simulink model "w3_warplab_buffers"  (Simulink 7.7)
settings: Solver=VariableStepDiscrete  SolverMode=SingleTasking  StartTime=0.0  StopTime=100  RelTol=1e-3
InitFcn:
  | w3_warplab_buffers_init
StartFcn:
  | w3_warplab_buffers_init
values from neighbouring files (symbols this model uses):
  NumSamps_Rx_IQ = 2^15    (= 32768)    [w3_warplab_buffers_init.m]
  NumSamps_Rx_RSSI = 2^13    (= 8192)    [w3_warplab_buffers_init.m]
  NumSamps_Tx_IQ = 2^15    (= 32768)    [w3_warplab_buffers_init.m]
undefined symbols (not defined in the file or in its folder): gcbh, xlBlockLoadCallback, xlGetNormalizedPeriod
libraries: xbsIndex_r4 x453, xbsEDKLib_r4 x1
(part 2 of 5)

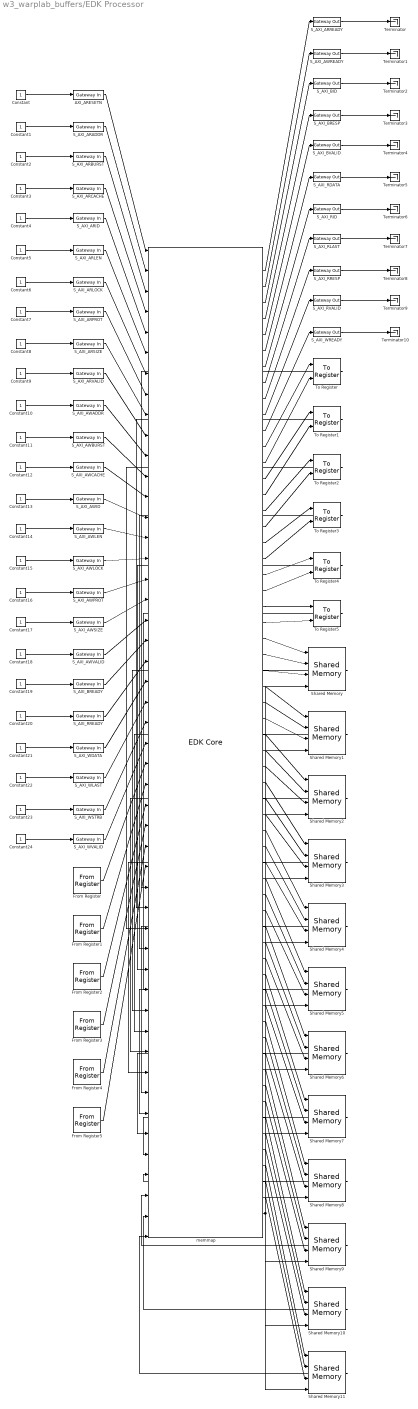
== system w3_warplab_buffers/EDK Processor ==
  AXI_ARESETN : xbsIndex_r4/Gateway In  gui_display_data_type=Fixed-point  arith_type=Boolean  n_bits=16  bin_pt=14  preci_type=Single  exp_width=8  frac_width=24  quantization="Round  (unbiased: +/- Inf)"  overflow=Saturate  period=xlGetNormalizedPeriod()  dbl_ovrd=off  timing_constraint=None  locs_specified=off  LOCs={}  UseAsADC=off  ADCChannel='1'  inherit_from_input=off  hdl_port=on  block_type=gatewayin
  Constant{,1..24} (25 alike) : Constant
  From Register : xbsIndex_r4/From Register  shared_memory_name='BUFF_SIZES'  init=0  period=xlGetNormalizedPeriod()  ownership=Owned and initialized elsewhere  gui_display_data_type=Fixed-point  arith_type=Unsigned  n_bits=32  bin_pt=0  preci_type=Single  dbl_ovrd=off  block_type=fromreg
      settings: AttributesFormatString=<< %<shared_memory_name> >>  infoedit="Register block that reads data to a shared memory register.  Delay of one sample period."
  From Register1 : xbsIndex_r4/From Register  shared_memory_name='DESIGN_VER'  init=0  period=xlGetNormalizedPeriod()  ownership=Owned and initialized elsewhere  gui_display_data_type=Fixed-point  arith_type=Unsigned  n_bits=32  bin_pt=0  preci_type=Single  dbl_ovrd=off  block_type=fromreg
      settings: AttributesFormatString=<< %<shared_memory_name> >>  infoedit="Register block that reads data to a shared memory register.  Delay of one sample period."
  From Register2 : xbsIndex_r4/From Register  shared_memory_name='STATUS'  init=0  period=xlGetNormalizedPeriod()  ownership=Owned and initialized elsewhere  gui_display_data_type=Fixed-point  arith_type=Unsigned  n_bits=2  bin_pt=0  preci_type=Single  dbl_ovrd=off  block_type=fromreg
      settings: AttributesFormatString=<< %<shared_memory_name> >>  infoedit="Register block that reads data to a shared memory register.  Delay of one sample period."
  From Register3 : xbsIndex_r4/From Register  shared_memory_name='RFCD_AGCDoneRSSI'  init=0  period=xlGetNormalizedPeriod()  ownership=Owned and initialized elsewhere  gui_display_data_type=Fixed-point  arith_type=Unsigned  n_bits=32  bin_pt=0  preci_type=Single  dbl_ovrd=off  block_type=fromreg
      settings: AttributesFormatString=<< %<shared_memory_name> >>  infoedit="Register block that reads data to a shared memory register.  Delay of one sample period."
  From Register4 : xbsIndex_r4/From Register  shared_memory_name='RFAB_AGCDoneRSSI'  init=0  period=xlGetNormalizedPeriod()  ownership=Owned and initialized elsewhere  gui_display_data_type=Fixed-point  arith_type=Unsigned  n_bits=32  bin_pt=0  preci_type=Single  dbl_ovrd=off  block_type=fromreg
      settings: AttributesFormatString=<< %<shared_memory_name> >>  infoedit="Register block that reads data to a shared memory register.  Delay of one sample period."
  From Register5 : xbsIndex_r4/From Register  shared_memory_name='AGCDoneAddr'  init=0  period=xlGetNormalizedPeriod()  ownership=Owned and initialized elsewhere  gui_display_data_type=Fixed-point  arith_type=Unsigned  n_bits=32  bin_pt=0  preci_type=Single  dbl_ovrd=off  block_type=fromreg
      settings: AttributesFormatString=<< %<shared_memory_name> >>  infoedit="Register block that reads data to a shared memory register.  Delay of one sample period."
  S_AXI_ARADDR : xbsIndex_r4/Gateway In  gui_display_data_type=Fixed-point  arith_type=Unsigned  n_bits=32  bin_pt=0  preci_type=Single  exp_width=8  frac_width=24  quantization="Round  (unbiased: +/- Inf)"  overflow=Saturate  period=xlGetNormalizedPeriod()  dbl_ovrd=off  timing_constraint=None  locs_specified=off  LOCs={}  UseAsADC=off  ADCChannel='1'  inherit_from_input=off  hdl_port=on  block_type=gatewayin
  S_AXI_ARBURST : xbsIndex_r4/Gateway In  gui_display_data_type=Fixed-point  arith_type=Unsigned  n_bits=2  bin_pt=0  preci_type=Single  exp_width=8  frac_width=24  quantization="Round  (unbiased: +/- Inf)"  overflow=Saturate  period=xlGetNormalizedPeriod()  dbl_ovrd=off  timing_constraint=None  locs_specified=off  LOCs={}  UseAsADC=off  ADCChannel='1'  inherit_from_input=off  hdl_port=on  block_type=gatewayin
  S_AXI_ARCACHE : xbsIndex_r4/Gateway In  gui_display_data_type=Fixed-point  arith_type=Unsigned  n_bits=4  bin_pt=0  preci_type=Single  exp_width=8  frac_width=24  quantization="Round  (unbiased: +/- Inf)"  overflow=Saturate  period=xlGetNormalizedPeriod()  dbl_ovrd=off  timing_constraint=None  locs_specified=off  LOCs={}  UseAsADC=off  ADCChannel='1'  inherit_from_input=off  hdl_port=on  block_type=gatewayin
  S_AXI_ARID : xbsIndex_r4/Gateway In  gui_display_data_type=Fixed-point  arith_type=Unsigned  n_bits=8  bin_pt=0  preci_type=Single  exp_width=8  frac_width=24  quantization="Round  (unbiased: +/- Inf)"  overflow=Saturate  period=xlGetNormalizedPeriod()  dbl_ovrd=off  timing_constraint=None  locs_specified=off  LOCs={}  UseAsADC=off  ADCChannel='1'  inherit_from_input=off  hdl_port=on  block_type=gatewayin
  S_AXI_ARLEN : xbsIndex_r4/Gateway In  gui_display_data_type=Fixed-point  arith_type=Unsigned  n_bits=8  bin_pt=0  preci_type=Single  exp_width=8  frac_width=24  quantization="Round  (unbiased: +/- Inf)"  overflow=Saturate  period=xlGetNormalizedPeriod()  dbl_ovrd=off  timing_constraint=None  locs_specified=off  LOCs={}  UseAsADC=off  ADCChannel='1'  inherit_from_input=off  hdl_port=on  block_type=gatewayin
  S_AXI_ARLOCK : xbsIndex_r4/Gateway In  gui_display_data_type=Fixed-point  arith_type=Unsigned  n_bits=2  bin_pt=0  preci_type=Single  exp_width=8  frac_width=24  quantization="Round  (unbiased: +/- Inf)"  overflow=Saturate  period=xlGetNormalizedPeriod()  dbl_ovrd=off  timing_constraint=None  locs_specified=off  LOCs={}  UseAsADC=off  ADCChannel='1'  inherit_from_input=off  hdl_port=on  block_type=gatewayin
  S_AXI_ARPROT : xbsIndex_r4/Gateway In  gui_display_data_type=Fixed-point  arith_type=Unsigned  n_bits=3  bin_pt=0  preci_type=Single  exp_width=8  frac_width=24  quantization="Round  (unbiased: +/- Inf)"  overflow=Saturate  period=xlGetNormalizedPeriod()  dbl_ovrd=off  timing_constraint=None  locs_specified=off  LOCs={}  UseAsADC=off  ADCChannel='1'  inherit_from_input=off  hdl_port=on  block_type=gatewayin
  S_AXI_ARREADY : xbsIndex_r4/Gateway Out  inherit_from_input=off  hdl_port=on  timing_constraint=None  locs_specified=off  LOCs={}  UseAsDAC=off  DACChannel='1'  block_type=gatewayout
  S_AXI_ARSIZE : xbsIndex_r4/Gateway In  gui_display_data_type=Fixed-point  arith_type=Unsigned  n_bits=3  bin_pt=0  preci_type=Single  exp_width=8  frac_width=24  quantization="Round  (unbiased: +/- Inf)"  overflow=Saturate  period=xlGetNormalizedPeriod()  dbl_ovrd=off  timing_constraint=None  locs_specified=off  LOCs={}  UseAsADC=off  ADCChannel='1'  inherit_from_input=off  hdl_port=on  block_type=gatewayin
  S_AXI_ARVALID : xbsIndex_r4/Gateway In  gui_display_data_type=Fixed-point  arith_type=Boolean  n_bits=16  bin_pt=14  preci_type=Single  exp_width=8  frac_width=24  quantization="Round  (unbiased: +/- Inf)"  overflow=Saturate  period=xlGetNormalizedPeriod()  dbl_ovrd=off  timing_constraint=None  locs_specified=off  LOCs={}  UseAsADC=off  ADCChannel='1'  inherit_from_input=off  hdl_port=on  block_type=gatewayin
  S_AXI_AWADDR : xbsIndex_r4/Gateway In  gui_display_data_type=Fixed-point  arith_type=Unsigned  n_bits=32  bin_pt=0  preci_type=Single  exp_width=8  frac_width=24  quantization="Round  (unbiased: +/- Inf)"  overflow=Saturate  period=xlGetNormalizedPeriod()  dbl_ovrd=off  timing_constraint=None  locs_specified=off  LOCs={}  UseAsADC=off  ADCChannel='1'  inherit_from_input=off  hdl_port=on  block_type=gatewayin
  S_AXI_AWBURST : xbsIndex_r4/Gateway In  gui_display_data_type=Fixed-point  arith_type=Unsigned  n_bits=2  bin_pt=0  preci_type=Single  exp_width=8  frac_width=24  quantization="Round  (unbiased: +/- Inf)"  overflow=Saturate  period=xlGetNormalizedPeriod()  dbl_ovrd=off  timing_constraint=None  locs_specified=off  LOCs={}  UseAsADC=off  ADCChannel='1'  inherit_from_input=off  hdl_port=on  block_type=gatewayin
  S_AXI_AWCACHE : xbsIndex_r4/Gateway In  gui_display_data_type=Fixed-point  arith_type=Unsigned  n_bits=4  bin_pt=0  preci_type=Single  exp_width=8  frac_width=24  quantization="Round  (unbiased: +/- Inf)"  overflow=Saturate  period=xlGetNormalizedPeriod()  dbl_ovrd=off  timing_constraint=None  locs_specified=off  LOCs={}  UseAsADC=off  ADCChannel='1'  inherit_from_input=off  hdl_port=on  block_type=gatewayin
  S_AXI_AWID : xbsIndex_r4/Gateway In  gui_display_data_type=Fixed-point  arith_type=Unsigned  n_bits=8  bin_pt=0  preci_type=Single  exp_width=8  frac_width=24  quantization="Round  (unbiased: +/- Inf)"  overflow=Saturate  period=xlGetNormalizedPeriod()  dbl_ovrd=off  timing_constraint=None  locs_specified=off  LOCs={}  UseAsADC=off  ADCChannel='1'  inherit_from_input=off  hdl_port=on  block_type=gatewayin
  S_AXI_AWLEN : xbsIndex_r4/Gateway In  gui_display_data_type=Fixed-point  arith_type=Unsigned  n_bits=8  bin_pt=0  preci_type=Single  exp_width=8  frac_width=24  quantization="Round  (unbiased: +/- Inf)"  overflow=Saturate  period=xlGetNormalizedPeriod()  dbl_ovrd=off  timing_constraint=None  locs_specified=off  LOCs={}  UseAsADC=off  ADCChannel='1'  inherit_from_input=off  hdl_port=on  block_type=gatewayin
  S_AXI_AWLOCK : xbsIndex_r4/Gateway In  gui_display_data_type=Fixed-point  arith_type=Unsigned  n_bits=2  bin_pt=0  preci_type=Single  exp_width=8  frac_width=24  quantization="Round  (unbiased: +/- Inf)"  overflow=Saturate  period=xlGetNormalizedPeriod()  dbl_ovrd=off  timing_constraint=None  locs_specified=off  LOCs={}  UseAsADC=off  ADCChannel='1'  inherit_from_input=off  hdl_port=on  block_type=gatewayin
  S_AXI_AWPROT : xbsIndex_r4/Gateway In  gui_display_data_type=Fixed-point  arith_type=Unsigned  n_bits=3  bin_pt=0  preci_type=Single  exp_width=8  frac_width=24  quantization="Round  (unbiased: +/- Inf)"  overflow=Saturate  period=xlGetNormalizedPeriod()  dbl_ovrd=off  timing_constraint=None  locs_specified=off  LOCs={}  UseAsADC=off  ADCChannel='1'  inherit_from_input=off  hdl_port=on  block_type=gatewayin
  S_AXI_AWREADY : xbsIndex_r4/Gateway Out  inherit_from_input=off  hdl_port=on  timing_constraint=None  locs_specified=off  LOCs={}  UseAsDAC=off  DACChannel='1'  block_type=gatewayout
  S_AXI_AWSIZE : xbsIndex_r4/Gateway In  gui_display_data_type=Fixed-point  arith_type=Unsigned  n_bits=3  bin_pt=0  preci_type=Single  exp_width=8  frac_width=24  quantization="Round  (unbiased: +/- Inf)"  overflow=Saturate  period=xlGetNormalizedPeriod()  dbl_ovrd=off  timing_constraint=None  locs_specified=off  LOCs={}  UseAsADC=off  ADCChannel='1'  inherit_from_input=off  hdl_port=on  block_type=gatewayin
  S_AXI_AWVALID : xbsIndex_r4/Gateway In  gui_display_data_type=Fixed-point  arith_type=Boolean  n_bits=16  bin_pt=14  preci_type=Single  exp_width=8  frac_width=24  quantization="Round  (unbiased: +/- Inf)"  overflow=Saturate  period=xlGetNormalizedPeriod()  dbl_ovrd=off  timing_constraint=None  locs_specified=off  LOCs={}  UseAsADC=off  ADCChannel='1'  inherit_from_input=off  hdl_port=on  block_type=gatewayin
  S_AXI_BID : xbsIndex_r4/Gateway Out  inherit_from_input=off  hdl_port=on  timing_constraint=None  locs_specified=off  LOCs={}  UseAsDAC=off  DACChannel='1'  block_type=gatewayout
  S_AXI_BREADY : xbsIndex_r4/Gateway In  gui_display_data_type=Fixed-point  arith_type=Boolean  n_bits=16  bin_pt=14  preci_type=Single  exp_width=8  frac_width=24  quantization="Round  (unbiased: +/- Inf)"  overflow=Saturate  period=xlGetNormalizedPeriod()  dbl_ovrd=off  timing_constraint=None  locs_specified=off  LOCs={}  UseAsADC=off  ADCChannel='1'  inherit_from_input=off  hdl_port=on  block_type=gatewayin
  S_AXI_BRESP : xbsIndex_r4/Gateway Out  inherit_from_input=off  hdl_port=on  timing_constraint=None  locs_specified=off  LOCs={}  UseAsDAC=off  DACChannel='1'  block_type=gatewayout
  S_AXI_BVALID : xbsIndex_r4/Gateway Out  inherit_from_input=off  hdl_port=on  timing_constraint=None  locs_specified=off  LOCs={}  UseAsDAC=off  DACChannel='1'  block_type=gatewayout
  S_AXI_RDATA : xbsIndex_r4/Gateway Out  inherit_from_input=off  hdl_port=on  timing_constraint=None  locs_specified=off  LOCs={}  UseAsDAC=off  DACChannel='1'  block_type=gatewayout
  S_AXI_RID : xbsIndex_r4/Gateway Out  inherit_from_input=off  hdl_port=on  timing_constraint=None  locs_specified=off  LOCs={}  UseAsDAC=off  DACChannel='1'  block_type=gatewayout
  S_AXI_RLAST : xbsIndex_r4/Gateway Out  inherit_from_input=off  hdl_port=on  timing_constraint=None  locs_specified=off  LOCs={}  UseAsDAC=off  DACChannel='1'  block_type=gatewayout
  S_AXI_RREADY : xbsIndex_r4/Gateway In  gui_display_data_type=Fixed-point  arith_type=Boolean  n_bits=16  bin_pt=14  preci_type=Single  exp_width=8  frac_width=24  quantization="Round  (unbiased: +/- Inf)"  overflow=Saturate  period=xlGetNormalizedPeriod()  dbl_ovrd=off  timing_constraint=None  locs_specified=off  LOCs={}  UseAsADC=off  ADCChannel='1'  inherit_from_input=off  hdl_port=on  block_type=gatewayin
  S_AXI_RRESP : xbsIndex_r4/Gateway Out  inherit_from_input=off  hdl_port=on  timing_constraint=None  locs_specified=off  LOCs={}  UseAsDAC=off  DACChannel='1'  block_type=gatewayout
  S_AXI_RVALID : xbsIndex_r4/Gateway Out  inherit_from_input=off  hdl_port=on  timing_constraint=None  locs_specified=off  LOCs={}  UseAsDAC=off  DACChannel='1'  block_type=gatewayout
  S_AXI_WDATA : xbsIndex_r4/Gateway In  gui_display_data_type=Fixed-point  arith_type=Unsigned  n_bits=32  bin_pt=0  preci_type=Single  exp_width=8  frac_width=24  quantization="Round  (unbiased: +/- Inf)"  overflow=Saturate  period=xlGetNormalizedPeriod()  dbl_ovrd=off  timing_constraint=None  locs_specified=off  LOCs={}  UseAsADC=off  ADCChannel='1'  inherit_from_input=off  hdl_port=on  block_type=gatewayin
  S_AXI_WLAST : xbsIndex_r4/Gateway In  gui_display_data_type=Fixed-point  arith_type=Boolean  n_bits=16  bin_pt=14  preci_type=Single  exp_width=8  frac_width=24  quantization="Round  (unbiased: +/- Inf)"  overflow=Saturate  period=xlGetNormalizedPeriod()  dbl_ovrd=off  timing_constraint=None  locs_specified=off  LOCs={}  UseAsADC=off  ADCChannel='1'  inherit_from_input=off  hdl_port=on  block_type=gatewayin
  S_AXI_WREADY : xbsIndex_r4/Gateway Out  inherit_from_input=off  hdl_port=on  timing_constraint=None  locs_specified=off  LOCs={}  UseAsDAC=off  DACChannel='1'  block_type=gatewayout
  S_AXI_WSTRB : xbsIndex_r4/Gateway In  gui_display_data_type=Fixed-point  arith_type=Unsigned  n_bits=4  bin_pt=0  preci_type=Single  exp_width=8  frac_width=24  quantization="Round  (unbiased: +/- Inf)"  overflow=Saturate  period=xlGetNormalizedPeriod()  dbl_ovrd=off  timing_constraint=None  locs_specified=off  LOCs={}  UseAsADC=off  ADCChannel='1'  inherit_from_input=off  hdl_port=on  block_type=gatewayin
  S_AXI_WVALID : xbsIndex_r4/Gateway In  gui_display_data_type=Fixed-point  arith_type=Boolean  n_bits=16  bin_pt=14  preci_type=Single  exp_width=8  frac_width=24  quantization="Round  (unbiased: +/- Inf)"  overflow=Saturate  period=xlGetNormalizedPeriod()  dbl_ovrd=off  timing_constraint=None  locs_specified=off  LOCs={}  UseAsADC=off  ADCChannel='1'  inherit_from_input=off  hdl_port=on  block_type=gatewayin
  Shared Memory : xbsIndex_r4/Shared Memory  shared_memory_name='RFD_IQ_Tx_Buffer'  depth=32768  ownership=Owned and Initialized Elsewhere  initVector=sin(pi*(0:15)/16)  en=on  mutex=Unprotected  mode=Read and Write  write_mode=Read Before Write  time_out=0  latency=1  explicit_data_type=off  gui_display_data_type=Fixed-point  arith_type=Unsigned  n_bits=32  bin_pt=0  preci_type=Single  implementation=Block RAM  use_rpm=off  block_type=shmem
      settings: AttributesFormatString=<< %<shared_memory_name> >>
  Shared Memory1 : xbsIndex_r4/Shared Memory  shared_memory_name='RFD_RSSI_Buffer'  depth=4096  ownership=Owned and Initialized Elsewhere  initVector=sin(pi*(0:15)/16)  en=on  mutex=Unprotected  mode=Read and Write  write_mode=Read Before Write  time_out=0  latency=1  explicit_data_type=off  gui_display_data_type=Fixed-point  arith_type=Unsigned  n_bits=32  bin_pt=0  preci_type=Single  implementation=Block RAM  use_rpm=off  block_type=shmem
      settings: AttributesFormatString=<< %<shared_memory_name> >>
  Shared Memory10 : xbsIndex_r4/Shared Memory  shared_memory_name='RFA_RSSI_Buffer'  depth=4096  ownership=Owned and Initialized Elsewhere  initVector=sin(pi*(0:15)/16)  en=on  mutex=Unprotected  mode=Read and Write  write_mode=Read Before Write  time_out=0  latency=1  explicit_data_type=off  gui_display_data_type=Fixed-point  arith_type=Unsigned  n_bits=32  bin_pt=0  preci_type=Single  implementation=Block RAM  use_rpm=off  block_type=shmem
      settings: AttributesFormatString=<< %<shared_memory_name> >>
  Shared Memory11 : xbsIndex_r4/Shared Memory  shared_memory_name='RFA_IQ_Rx_Buffer'  depth=32768  ownership=Owned and Initialized Elsewhere  initVector=sin(pi*(0:15)/16)  en=on  mutex=Unprotected  mode=Read and Write  write_mode=Read Before Write  time_out=0  latency=1  explicit_data_type=off  gui_display_data_type=Fixed-point  arith_type=Unsigned  n_bits=32  bin_pt=0  preci_type=Single  implementation=Block RAM  use_rpm=off  block_type=shmem
      settings: AttributesFormatString=<< %<shared_memory_name> >>
  Shared Memory2 : xbsIndex_r4/Shared Memory  shared_memory_name='RFD_IQ_Rx_Buffer'  depth=32768  ownership=Owned and Initialized Elsewhere  initVector=sin(pi*(0:15)/16)  en=on  mutex=Unprotected  mode=Read and Write  write_mode=Read Before Write  time_out=0  latency=1  explicit_data_type=off  gui_display_data_type=Fixed-point  arith_type=Unsigned  n_bits=32  bin_pt=0  preci_type=Single  implementation=Block RAM  use_rpm=off  block_type=shmem
      settings: AttributesFormatString=<< %<shared_memory_name> >>
  Shared Memory3 : xbsIndex_r4/Shared Memory  shared_memory_name='RFC_IQ_Tx_Buffer'  depth=32768  ownership=Owned and Initialized Elsewhere  initVector=sin(pi*(0:15)/16)  en=on  mutex=Unprotected  mode=Read and Write  write_mode=Read Before Write  time_out=0  latency=1  explicit_data_type=off  gui_display_data_type=Fixed-point  arith_type=Unsigned  n_bits=32  bin_pt=0  preci_type=Single  implementation=Block RAM  use_rpm=off  block_type=shmem
      settings: AttributesFormatString=<< %<shared_memory_name> >>
  Shared Memory4 : xbsIndex_r4/Shared Memory  shared_memory_name='RFC_RSSI_Buffer'  depth=4096  ownership=Owned and Initialized Elsewhere  initVector=sin(pi*(0:15)/16)  en=on  mutex=Unprotected  mode=Read and Write  write_mode=Read Before Write  time_out=0  latency=1  explicit_data_type=off  gui_display_data_type=Fixed-point  arith_type=Unsigned  n_bits=32  bin_pt=0  preci_type=Single  implementation=Block RAM  use_rpm=off  block_type=shmem
      settings: AttributesFormatString=<< %<shared_memory_name> >>
  Shared Memory5 : xbsIndex_r4/Shared Memory  shared_memory_name='RFC_IQ_Rx_Buffer'  depth=32768  ownership=Owned and Initialized Elsewhere  initVector=sin(pi*(0:15)/16)  en=on  mutex=Unprotected  mode=Read and Write  write_mode=Read Before Write  time_out=0  latency=1  explicit_data_type=off  gui_display_data_type=Fixed-point  arith_type=Unsigned  n_bits=32  bin_pt=0  preci_type=Single  implementation=Block RAM  use_rpm=off  block_type=shmem
      settings: AttributesFormatString=<< %<shared_memory_name> >>
  Shared Memory6 : xbsIndex_r4/Shared Memory  shared_memory_name='RFB_IQ_Tx_Buffer'  depth=32768  ownership=Owned and Initialized Elsewhere  initVector=sin(pi*(0:15)/16)  en=on  mutex=Unprotected  mode=Read and Write  write_mode=Read Before Write  time_out=0  latency=1  explicit_data_type=off  gui_display_data_type=Fixed-point  arith_type=Unsigned  n_bits=32  bin_pt=0  preci_type=Single  implementation=Block RAM  use_rpm=off  block_type=shmem
      settings: AttributesFormatString=<< %<shared_memory_name> >>
  Shared Memory7 : xbsIndex_r4/Shared Memory  shared_memory_name='RFB_RSSI_Buffer'  depth=4096  ownership=Owned and Initialized Elsewhere  initVector=sin(pi*(0:15)/16)  en=on  mutex=Unprotected  mode=Read and Write  write_mode=Read Before Write  time_out=0  latency=1  explicit_data_type=off  gui_display_data_type=Fixed-point  arith_type=Unsigned  n_bits=32  bin_pt=0  preci_type=Single  implementation=Block RAM  use_rpm=off  block_type=shmem
      settings: AttributesFormatString=<< %<shared_memory_name> >>
  Shared Memory8 : xbsIndex_r4/Shared Memory  shared_memory_name='RFB_IQ_Rx_Buffer'  depth=32768  ownership=Owned and Initialized Elsewhere  initVector=sin(pi*(0:15)/16)  en=on  mutex=Unprotected  mode=Read and Write  write_mode=Read Before Write  time_out=0  latency=1  explicit_data_type=off  gui_display_data_type=Fixed-point  arith_type=Unsigned  n_bits=32  bin_pt=0  preci_type=Single  implementation=Block RAM  use_rpm=off  block_type=shmem
      settings: AttributesFormatString=<< %<shared_memory_name> >>
  Shared Memory9 : xbsIndex_r4/Shared Memory  shared_memory_name='RFA_IQ_Tx_Buffer'  depth=32768  ownership=Owned and Initialized Elsewhere  initVector=sin(pi*(0:15)/16)  en=on  mutex=Unprotected  mode=Read and Write  write_mode=Read Before Write  time_out=0  latency=1  explicit_data_type=off  gui_display_data_type=Fixed-point  arith_type=Unsigned  n_bits=32  bin_pt=0  preci_type=Single  implementation=Block RAM  use_rpm=off  block_type=shmem
      settings: AttributesFormatString=<< %<shared_memory_name> >>
  Terminator{,1..10} (11 alike) : Terminator
  To Register : xbsIndex_r4/To Register  shared_memory_name='TxDelay'  init=0  ownership=Owned and initialized elsewhere  explicit_data_type=on  gui_display_data_type=Fixed-point  arith_type=Unsigned  n_bits=32  bin_pt=0  preci_type=Single  dbl_ovrd=off  block_type=toreg
      settings: AttributesFormatString=<< %<shared_memory_name> >>  infoedit="Register block that writes data to a shared memory register.  Delay of one sample period."
  To Register1 : xbsIndex_r4/To Register  shared_memory_name='RX_BUFF_EN'  init=0  ownership=Owned and initialized elsewhere  explicit_data_type=on  gui_display_data_type=Fixed-point  arith_type=Unsigned  n_bits=32  bin_pt=0  preci_type=Single  dbl_ovrd=off  block_type=toreg
      settings: AttributesFormatString=<< %<shared_memory_name> >>  infoedit="Register block that writes data to a shared memory register.  Delay of one sample period."
  To Register2 : xbsIndex_r4/To Register  shared_memory_name='CONFIG'  init=0  ownership=Owned and initialized elsewhere  explicit_data_type=on  gui_display_data_type=Fixed-point  arith_type=Unsigned  n_bits=32  bin_pt=0  preci_type=Single  dbl_ovrd=off  block_type=toreg
      settings: AttributesFormatString=<< %<shared_memory_name> >>  infoedit="Register block that writes data to a shared memory register.  Delay of one sample period."
  To Register3 : xbsIndex_r4/To Register  shared_memory_name='TX_BUFF_EN'  init=0  ownership=Owned and initialized elsewhere  explicit_data_type=on  gui_display_data_type=Fixed-point  arith_type=Unsigned  n_bits=32  bin_pt=0  preci_type=Single  dbl_ovrd=off  block_type=toreg
      settings: AttributesFormatString=<< %<shared_memory_name> >>  infoedit="Register block that writes data to a shared memory register.  Delay of one sample period."
  To Register4 : xbsIndex_r4/To Register  shared_memory_name='RxLength'  init=0  ownership=Owned and initialized elsewhere  explicit_data_type=on  gui_display_data_type=Fixed-point  arith_type=Unsigned  n_bits=24  bin_pt=0  preci_type=Single  dbl_ovrd=off  block_type=toreg
      settings: AttributesFormatString=<< %<shared_memory_name> >>  infoedit="Register block that writes data to a shared memory register.  Delay of one sample period."
  To Register5 : xbsIndex_r4/To Register  shared_memory_name='TxLength'  init=0  ownership=Owned and initialized elsewhere  explicit_data_type=on  gui_display_data_type=Fixed-point  arith_type=Unsigned  n_bits=24  bin_pt=0  preci_type=Single  dbl_ovrd=off  block_type=toreg
      settings: AttributesFormatString=<< %<shared_memory_name> >>  infoedit="Register block that writes data to a shared memory register.  Delay of one sample period."
  memmap : xbsEDKLib_r4/EDK Core  sim_method=Inactive  xmp=xmp  blockname=blockname  dual_clock=dual_clock  procinfo=procinfo  bus_type=bus_type  memxtable=memxtable  memmap_hdlcontent=|  config={'inports'=>[{'arith_type'=>2.00000000000000000,'bin_pt'=>0.00000000000000000,'name'=>'AXI_ARESETN','width'=>0},{'arith_type'=>2.00000000000000000,'bin_pt'=>0.00000000000000000,'name'=>'S_AXI_ARADDR','width'=>32},{'arith_type'=>2.00000000000000000,'bin_pt'=>0.00000000000000000,'name'=>'S_AXI_ARBURST','width'=>2},{'arith_type'=>2.00000000000000000,'bin_pt'=>0.00000000000000000,'name'=>'S_AXI_ARCACHE','width'=>4},{'arith_type'=>2.00000000000000000,'bin_pt'=>0.00000000000000000,'name'=>'S_AXI_ARID','width'=>8},{'arith_type'=>2.00000000000000000,'bin_pt'=>0.00000000000000000,'name'=>'S_AXI_ARLEN','width'=>8},{'arith_type'=>2.00000000000000000,'bin_pt'=>0.00000000000000000,'name'=>'S_AXI_ARLOCK','width'=>2},{'arith_type'=>2.00000000000000000,'bin_pt'=>0.00000000000000000,'name'=>'S_AXI_ARPROT','width'=>3},{'arith_type'=>2.00000000000000000,'bin_pt'=>0.00000000000000000,'name'=>'S_AXI_ARSIZE','width'=>3},{'arith_type'=>2.00000000000000000,'bin_pt'=>0.00000000000000000,'name'=>'S_AXI_ARVALID','width'=>0},{'arith_type'=>2.00000000000000000,'bin_pt'=>0.00000000000000000,'name'=>'S_AXI_AWADDR','width'=>32},{'arith_type'=>2.00000000000000000,'bin_pt'=>0.00000000000000000,'name'=>'S_AXI_AWBURST','width'=>2},{'arith_type'=>2.00000000000000000,'bin_pt'=>0.00000000000000000,'name'=>'S_AXI_AWCACHE','width'=>4},{'arith_type'=>2.00000000000000000,'bin_pt'=>0.00000000000000000,'name'=>'S_AXI_AWID','width'=>8},{'arith_type'=>2.00000000000000000,'bin_pt'=>0.00000000000000000,'name'=>'S_AXI_AWLEN','width'=>8},{'arith_type'=>2.00000000000000000,'bin_pt'=>0.00000000000000000,'name'=>'S_AXI_AWLOCK','width'=>2},{'arith_type'=>2.00000000000000000,'bin_pt'=>0.00000000000000000,'name'=>'S_AXI_AWPROT','width'=>3},{'arith_type'=>2.00000000000000000,'bin_pt'=>0.00000000000000000,'name'=>'S_AXI_AWSIZE','width'=>3},{'arith_type'=>2.00000000000000000,'bin_pt'=>0.00000000000000000,'name'=>'S_AXI_AWVALID','width'=>0},{'arith_type'=>2.00000000000000000,'bin_pt'=>0.00000000000000000,'name'=>'S_AXI_BREADY','width'=>0},{'arith_type'=>2.00000000000000000,'bin_pt'=>0.00000000000000000,'name'=>'S_AXI_RREADY','width'=>0},{'arith_type'=>2.00000000000000000,'bin_pt'=>0.00000000000000000,'name'=>'S_AXI_WDATA','width'=>32},{'arith_type'=>2.00000000000000000,'bin_pt'=>0.00000000000000000,'name'=>'S_AXI_WLAST','width'=>0},{'arith_type'=>2.00000000000000000,'bin_pt'=>0.00000000000000000,'name'=>'S_AXI_WSTRB','width'=>4},{'arith_type'=>2.00000000000000000,'bin_pt'=>0.00000000000000000,'name'=>'S_AXI_WVALID','width'=>0},{'arith_type'=>2,'bin_pt'=>0,'name'=>'sm_BUFF_SIZES_dout','width'=>32},{'arith_type'=>2,'bin_pt'=>0,'name'=>'sm_DESIGN_VER_dout','width'=>32},{'arith_type'=>2,'bin_pt'=>0,'name'=>'sm_STATUS_dout','width'=>2},{'arith_type'=>2,'bin_pt'=>0,'name'=>'sm_RFCD_AGCDoneRSSI_dout','width'=>32},{'arith_type'=>2,'bin_pt'=>0,'name'=>'sm_RFAB_AGCDoneRSSI_dout','width'=>32},{'arith_type'=>2,'bin_pt'=>0,'name'=>'sm_AGCDoneAddr_dout','width'=>32},{'arith_type'=>2,'bin_pt'=>0,'name'=>'sm_TxDelay_dout','width'=>32},{'arith_type'=>2,'bin_pt'=>0,'name'=>'sm_RX_BUFF_EN_dout','width'=>32},{'arith_type'=>2,'bin_pt'=>0,'name'=>'sm_CONFIG_dout','width'=>32},{'arith_type'=>2,'bin_pt'=>0,'name'=>'sm_TX_BUFF_EN_dout','width'=>32},{'arith_type'=>2,'bin_pt'=>0,'name'=>'sm_RxLength_dout','width'=>24},{'arith_type'=>2,'bin_pt'=>0,'name'=>'sm_TxLength_dout','width'=>24},{'arith_type'=>2,'bin_pt'=>0,'name'=>'sm_RFD_IQ_Tx_Buffer_dout','width'=>32},{'arith_type'=>2,'bin_pt'=>0,'name'=>'sm_RFD_RSSI_Buffer_dout','width'=>32},{'arith_type'=>2,'bin_pt'=>0,'name'=>'sm_RFD_IQ_Rx_Buffer_dout','width'=>32},{'arith_type'=>2,'bin_pt'=>0,'name'=>'sm_RFC_IQ_Tx_Buffer_dout','width'=>32},{'arith_type'=>2,'bin_pt'=>0,'name'=>'sm_RFC_RSSI_Buffer_dout','width'=>32},{'arith_type'=>2,'bin_pt'=>0,'name'=>'sm_RFC_IQ_Rx_Buffer_dout','width'=>32},{'arith_type'=>2,'bin_pt'=>0,'name'=>'sm_RFB_IQ_Tx_Buffer_dout','width'=>32},{'arith_type'=>2,'bin_pt'=>0,'name'=>'sm_RFB_RSSI_Buffer_dout','width'=>32},{'arith_type'=>2,'bin_pt'=>0,'name'=>'sm_RFB_IQ_Rx_Buffer_dout','width'=>32},{'arith_type'=>2,'bin_pt'=>0,'name'=>'sm_RFA_IQ_Tx_Buffer_dout','width'=>32},{'arith_type'=>2,'bin_pt'=>0,'name'=>'sm_RFA_RSSI_Buffer_dout','width'=>32},{'arith_type'=>2,'bin_pt'=>0,'name'=>'sm_RFA_IQ_Rx_Buffer_dout','width'=>32}],'outports'=>[{'arith_type'=>2.00000000000000000,'bin_pt'=>0.00000000000000000,'name'=>'S_AXI_ARREADY','width'=>0},{'arith_type'=>2.00000000000000000,'bin_pt'=>0.00000000000000000,'name'=>'S_AXI_AWREADY','width'=>0},{'arith_type'=>2.00000000000000000,'bin_pt'=>0.00000000000000000,'name'=>'S_AXI_BID','width'=>8},{'arith_type'=>2.00000000000000000,'bin_pt'=>0.00000000000000000,'name'=>'S_AXI_BRESP','width'=>2},{'arith_type'=>2.00000000000000000,'bin_pt'=>0.00000000000000000,'name'=>'S_AXI_BVALID','width'=>0},{'arith_type'=>2.00000000000000000,'bin_pt'=>0.00000000000000000,'name'=>'S_AXI_RDATA','width'=>32},{'arith_type'=>2.00000000000000000,'bin_pt'=>0.00000000000000000,'name'=>'S_AXI_RID','width'=>8},{'arith_type'=>2.00000000000000000,'bin_pt'=>0.00000000000000000,'name'=>'S_AXI_RLAST','width'=>0},{'arith_type'=>2.00000000000000000,'bin_pt'=>0.00000000000000000,'name'=>'S_AXI_RRESP','width'=>2},{'arith_type'=>2.00000000000000000,'bin_pt'=>0.00000000000000000,'name'=>'S_AXI_RVALID','width'=>0},{'arith_type'=>2.00000000000000000,'bin_pt'=>0.00000000000000000,'name'=>'S_AXI_WREADY','width'=>0},{'arith_type'=>2,'bin_pt'=>0,'name'=>'sm_TxDelay_din','width'=>32},{'arith_type'=>2.00000000000000000,'bin_pt'=>0.00000000000000000,'name'=>'sm_TxDelay_en','width'=>0.00000000000000000},{'arith_type'=>2,'bin_pt'=>0,'name'=>'sm_RX_BUFF_EN_din','width'=>32},{'arith_type'=>2.00000000000000000,'bin_pt'=>0.00000000000000000,'name'=>'sm_RX_BUFF_EN_en','width'=>0.00000000000000000},{'arith_type'=>2,'bin_pt'=>0,'name'=>'sm_CONFIG_din','width'=>32},{'arith_type'=>2.00000000000000000,'bin_pt'=>0.00000000000000000,'name'=>'sm_CONFIG_en','width'=>0.00000000000000000},{'arith_type'=>2,'bin_pt'=>0,'name'=>'sm_TX_BUFF_EN_din','width'=>32},{'arith_type'=>2.00000000000000000,'bin_pt'=>0.00000000000000000,'name'=>'sm_TX_BUFF_EN_en','width'=>0.00000000000000000},{'arith_type'=>2,'bin_pt'=>0,'name'=>'sm_RxLength_din','width'=>24},{'arith_type'=>2.00000000000000000,'bin_pt'=>0.00000000000000000,'name'=>'sm_RxLength_en','width'=>0.00000000000000000},{'arith_type'=>2,'bin_pt'=>0,'name'=>'sm_TxLength_din','width'=>24},{'arith_type'=>2.00000000000000000,'bin_pt'=>0.00000000000000000,'name'=>'sm_TxLength_en','width'=>0.00000000000000000},{'arith_type'=>2.00000000000000000,'bin_pt'=>0.00000000000000000,'name'=>'sm_RFD_IQ_Tx_Buffer_addr','width'=>15.00000000000000000},{'arith_type'=>2,'bin_pt'=>0,'name'=>'sm_RFD_IQ_Tx_Buffer_din','width'=>32},{'arith_type'=>2.00000000000000000,'bin_pt'=>0.00000000000000000,'name'=>'sm_RFD_IQ_Tx_Buffer_we','width'=>0.00000000000000000},{'arith_type'=>2.00000000000000000,'bin_pt'=>0.00000000000000000,'name'=>'sm_RFD_RSSI_Buffer_addr','width'=>12.00000000000000000},{'arith_type'=>2,'bin_pt'=>0,'name'=>'sm_RFD_RSSI_Buffer_din','width'=>32},{'arith_type'=>2.00000000000000000,'bin_pt'=>0.00000000000000000,'name'=>'sm_RFD_RSSI_Buffer_we','width'=>0.00000000000000000},{'arith_type'=>2.00000000000000000,'bin_pt'=>0.00000000000000000,'name'=>'sm_RFD_IQ_Rx_Buffer_addr','width'=>15.00000000000000000},{'arith_type'=>2,'bin_pt'=>0,'name'=>'sm_RFD_IQ_Rx_Buffer_din','width'=>32},{'arith_type'=>2.00000000000000000,'bin_pt'=>0.00000000000000000,'name'=>'sm_RFD_IQ_Rx_Buffer_we','width'=>0.00000000000000000},{'arith_type'=>2.00000000000000000,'bin_pt'=>0.00000000000000000,'name'=>'sm_RFC_IQ_Tx_Buffer_addr','width'=>15.00000000000000000},{'arith_type'=>2,'bin_pt'=>0,'name'=>'sm_RFC_IQ_Tx_Buffer_din','width'=>32},{'arith_type'=>2.00000000000000000,'bin_pt'=>0.00000000000000000,'name'=>'sm_RFC_IQ_Tx_Buffer_we','width'=>0.00000000000000000},{'arith_type'=>2.00000000000000000,'bin_pt'=>0.00000000000000000,'name'=>'sm_RFC_RSSI_Buffer_addr','width'=>12.00000000000000000},{'arith_type'=>2,'bin_pt'=>0,'name'=>'sm_RFC_RSSI_Buffer_din','width'=>32},{'arith_type'=>2.00000000000000000,'bin_pt'=>0.00000000000000000,'name'=>'sm_RFC_RSSI_Buffer_we','width'=>0.00000000000000000},{'arith_type'=>2.00000000000000000,'bin_pt'=>0.00000000000000000,'name'=>'sm_RFC_IQ_Rx_Buffer_addr','width'=>15.00000000000000000},{'arith_type'=>2,'bin_pt'=>0,'name'=>'sm_RFC_IQ_Rx_Buffer_din','width'=>32},{'arith_type'=>2.00000000000000000,'bin_pt'=>0.00000000000000000,'name'=>'sm_RFC_IQ_Rx_Buffer_we','width'=>0.00000000000000000},{'arith_type'=>2.00000000000000000,'bin_pt'=>0.00000000000000000,'name'=>'sm_RFB_IQ_Tx_Buffer_addr','width'=>15.00000000000000000},{'arith_type'=>2,'bin_pt'=>0,'name'=>'sm_RFB_IQ_Tx_Buffer_din','width'=>32},{'arith_type'=>2.00000000000000000,'bin_pt'=>0.00000000000000000,'name'=>'sm_RFB_IQ_Tx_Buffer_we','width'=>0.00000000000000000},{'arith_type'=>2.00000000000000000,'bin_pt'=>0.00000000000000000,'name'=>'sm_RFB_RSSI_Buffer_addr','width'=>12.00000000000000000},{'arith_type'=>2,'bin_pt'=>0,'name'=>'sm_RFB_RSSI_Buffer_din','width'=>32},{'arith_type'=>2.00000000000000000,'bin_pt'=>0.00000000000000000,'name'=>'sm_RFB_RSSI_Buffer_we','width'=>0.00000000000000000},{'arith_type'=>2.00000000000000000,'bin_pt'=>0.00000000000000000,'name'=>'sm_RFB_IQ_Rx_Buffer_addr','width'=>15.00000000000000000},{'arith_type'=>2,'bin_pt'=>0,'name'=>'sm_RFB_IQ_Rx_Buffer_din','width'=>32},{'arith_type'=>2.00000000000000000,'bin_pt'=>0.00000000000000000,'name'=>'sm_RFB_IQ_Rx_Buffer_we','width'=>0.00000000000000000},{'arith_type'=>2.00000000000000000,'bin_pt'=>0.00000000000000000,'name'=>'sm_RFA_IQ_Tx_Buffer_addr','width'=>15.00000000000000000},{'arith_type'=>2,'bin_pt'=>0,'name'=>'sm_RFA_IQ_Tx_Buffer_din','width'=>32},{'arith_type'=>2.00000000000000000,'bin_pt'=>0.00000000000000000,'name'=>'sm_RFA_IQ_Tx_Buffer_we','width'=>0.00000000000000000},{'arith_type'=>2.00000000000000000,'bin_pt'=>0.00000000000000000,'name'=>'sm_RFA_RSSI_Buffer_addr','width'=>12.00000000000000000},{'arith_type'=>2,'bin_pt'=>0,'name'=>'sm_RFA_RSSI_Buffer_din','width'=>32},{'arith_type'=>2.00000000000000000,'bin_pt'=>0.00000000000000000,'name'=>'sm_RFA_RSSI_Buffer_we','width'=>0.00000000000000000},{'arith_type'=>2.00000000000000000,'bin_pt'=>0.00000000000000000,'name'=>'sm_RFA_IQ_Rx_Buffer_addr','width'=>15.00000000000000000},{'arith_type'=>2,'bin_pt'=>0,'name'=>'sm_RFA_IQ_Rx_Buffer_din','width'=>32},{'arith_type'=>2.00000000000000000,'bin_pt'=>0.00000000000000000,'name'=>'sm_RFA_IQ_Rx_Buffer_we','width'=>0.00000000000000000},{'arith_type'=>1.00000000000000000,'bin_pt'=>0.00000000000000000,'name'=>'shram_en','width'=>0.00000000000000000}]}  inheritDeviceType=inheritDeviceType  block_type=edkcore
      | library IEEE;
      | use IEEE.std_logic_1164.all;
      | use IEEE.numeric_std.all;
      | 
      | entity axi_sgiface is
      |     generic (
      |         -- AXI specific.
      |         -- TODO: need to figure out a way to pass these generics from outside
      |         C_S_AXI_SUPPORT_BURST   : integer := 0;
      |         -- TODO: fix the internal ID width to 8
      |         C_S_AXI_ID_WIDTH        : integer := 8;
      |         C_S_AXI_DATA_WIDTH      : integer := 32;
      |         C_S_AXI_ADDR_WIDTH      : integer := 32;
      |         C_S_AXI_TOTAL_ADDR_LEN  : integer := 23;
      |         C_S_AXI_LINEAR_ADDR_LEN : integer := 19;
      |         C_S_AXI_BANK_ADDR_LEN   : integer := 2;
      |         C_S_AXI_AWLEN_WIDTH     : integer := 8;
      |         C_S_AXI_ARLEN_WIDTH     : integer := 8
      |     );
      |     port (
      |         -- General.
      |         AXI_AClk      : in  std_logic;
      |         AXI_AResetN    : in  std_logic;
      |         -- not used
      |         AXI_Ce        : in  std_logic;
      |   
      |         -- AXI Port.
      |         S_AXI_AWADDR  : in  std_logic_vector(C_S_AXI_ADDR_WIDTH-1 downto 0);
      |         S_AXI_AWID    : in  std_logic_vector(C_S_AXI_ID_WIDTH-1 downto 0);
      |         S_AXI_AWLEN   : in  std_logic_vector(C_S_AXI_AWLEN_WIDTH-1 downto 0);
      |         S_AXI_AWSIZE  : in  std_logic_vector(2 downto 0);
      |         S_AXI_AWBURST : in  std_logic_vector(1 downto 0);
      |         S_AXI_AWLOCK  : in  std_logic_vector(1 downto 0);
      |         S_AXI_AWCACHE : in  std_logic_vector(3 downto 0);
      |         S_AXI_AWPROT  : in  std_logic_vector(2 downto 0);
      |         S_AXI_AWVALID : in  std_logic;
      |         S_AXI_AWREADY : out std_logic;
      |         
      |         S_AXI_WLAST   : in  std_logic;
      |         S_AXI_WDATA   : in  std_logic_vector(C_S_AXI_DATA_WIDTH-1 downto 0);
      |         S_AXI_WSTRB   : in  std_logic_vector((C_S_AXI_DATA_WIDTH/8)-1 downto 0);
      |         S_AXI_WVALID  : in  std_logic;
      |         S_AXI_WREADY  : out std_logic;
      |         
      |         S_AXI_BRESP   : out std_logic_vector(1 downto 0);
      |         S_AXI_BID     : out std_logic_vector(C_S_AXI_ID_WIDTH-1 downto 0);
      |         S_AXI_BVALID  : out std_logic;
      |         S_AXI_BREADY  : in  std_logic;
      |         
      |         S_AXI_ARADDR  : in  std_logic_vector(C_S_AXI_ADDR_WIDTH-1 downto 0);
      |         S_AXI_ARID    : in  std_logic_vector(C_S_AXI_ID_WIDTH-1 downto 0);
      |         S_AXI_ARLEN   : in  std_logic_vector(C_S_AXI_ARLEN_WIDTH-1 downto 0);
      |         S_AXI_ARSIZE  : in  std_logic_vector(2 downto 0);
      |         S_AXI_ARBURST : in  std_logic_vector(1 downto 0);
      |         S_AXI_ARLOCK  : in  std_logic_vector(1 downto 0);
      |         S_AXI_ARCACHE : in  std_logic_vector(3 downto 0);
      |         S_AXI_ARPROT  : in  std_logic_vector(2 downto 0);
      |         S_AXI_ARVALID : in  std_logic;
      |         S_AXI_ARREADY : out std_logic;
      |         
      |         -- 'From Register'
      |         -- 'BUFF_SIZES'
      |         sm_BUFF_SIZES_dout : in std_logic_vector(32-1 downto 0);
      |         -- 'DESIGN_VER'
      |         sm_DESIGN_VER_dout : in std_logic_vector(32-1 downto 0);
      |         -- 'STATUS'
      |         sm_STATUS_dout : in std_logic_vector(2-1 downto 0);
      |         -- 'RFCD_AGCDoneRSSI'
      |         sm_RFCD_AGCDoneRSSI_dout : in std_logic_vector(32-1 downto 0);
      |         -- 'RFAB_AGCDoneRSSI'
      |         sm_RFAB_AGCDoneRSSI_dout : in std_logic_vector(32-1 downto 0);
      |         -- 'AGCDoneAddr'
      |         sm_AGCDoneAddr_dout : in std_logic_vector(32-1 downto 0);
      |         -- 'To Register'
      |         -- 'TxDelay'
      |         sm_TxDelay_dout : in std_logic_vector(32-1 downto 0);
      |         sm_TxDelay_din  : out std_logic_vector(32-1 downto 0);
      |         sm_TxDelay_en   : out std_logic;
      |         -- 'RX_BUFF_EN'
      |         sm_RX_BUFF_EN_dout : in std_logic_vector(32-1 downto 0);
      |         sm_RX_BUFF_EN_din  : out std_logic_vector(32-1 downto 0);
      |         sm_RX_BUFF_EN_en   : out std_logic;
      |         -- 'CONFIG'
      |         sm_CONFIG_dout : in std_logic_vector(32-1 downto 0);
      |         sm_CONFIG_din  : out std_logic_vector(32-1 downto 0);
      |         sm_CONFIG_en   : out std_logic;
      |         -- 'TX_BUFF_EN'
      |         sm_TX_BUFF_EN_dout : in std_logic_vector(32-1 downto 0);
      |         sm_TX_BUFF_EN_din  : out std_logic_vector(32-1 downto 0);
      |         sm_TX_BUFF_EN_en   : out std_logic;
      |         -- 'RxLength'
      |         sm_RxLength_dout : in std_logic_vector(24-1 downto 0);
      |         sm_RxLength_din  : out std_logic_vector(24-1 downto 0);
      |         sm_RxLength_en   : out std_logic;
      |         -- 'TxLength'
      |         sm_TxLength_dout : in std_logic_vector(24-1 downto 0);
      |         sm_TxLength_din  : out std_logic_vector(24-1 downto 0);
      |         sm_TxLength_en   : out std_logic;
      |         -- 'From FIFO'
      |         -- 'To FIFO'
      |         -- 'Shared Memory'
      |         -- 'RFD_IQ_Tx_Buffer'
      |         sm_RFD_IQ_Tx_Buffer_dout  : in  std_logic_vector(32-1 downto 0);
      |         sm_RFD_IQ_Tx_Buffer_addr  : out std_logic_vector(15-1 downto 0);
      |         sm_RFD_IQ_Tx_Buffer_din   : out std_logic_vector(32-1 downto 0);
      |         sm_RFD_IQ_Tx_Buffer_we    : out std_logic;
      |         -- 'RFD_RSSI_Buffer'
      |         sm_RFD_RSSI_Buffer_dout  : in  std_logic_vector(32-1 downto 0);
      |         sm_RFD_RSSI_Buffer_addr  : out std_logic_vector(12-1 downto 0);
      |         sm_RFD_RSSI_Buffer_din   : out std_logic_vector(32-1 downto 0);
      |         sm_RFD_RSSI_Buffer_we    : out std_logic;
      |         -- 'RFD_IQ_Rx_Buffer'
      |         sm_RFD_IQ_Rx_Buffer_dout  : in  std_logic_vector(32-1 downto 0);
      |         sm_RFD_IQ_Rx_Buffer_addr  : out std_logic_vector(15-1 downto 0);
      |         sm_RFD_IQ_Rx_Buffer_din   : out std_logic_vector(32-1 downto 0);
      |         sm_RFD_IQ_Rx_Buffer_we    : out std_logic;
      |         -- 'RFC_IQ_Tx_Buffer'
      |         sm_RFC_IQ_Tx_Buffer_dout  : in  std_logic_vector(32-1 downto 0);
      |         sm_RFC_IQ_Tx_Buffer_addr  : out std_logic_vector(15-1 downto 0);
      |         sm_RFC_IQ_Tx_Buffer_din   : out std_logic_vector(32-1 downto 0);
      |         sm_RFC_IQ_Tx_Buffer_we    : out std_logic;
      |         -- 'RFC_RSSI_Buffer'
      |         sm_RFC_RSSI_Buffer_dout  : in  std_logic_vector(32-1 downto 0);
      |         sm_RFC_RSSI_Buffer_addr  : out std_logic_vector(12-1 downto 0);
      |         sm_RFC_RSSI_Buffer_din   : out std_logic_vector(32-1 downto 0);
      |         sm_RFC_RSSI_Buffer_we    : out std_logic;
      |         -- 'RFC_IQ_Rx_Buffer'
      |         sm_RFC_IQ_Rx_Buffer_dout  : in  std_logic_vector(32-1 downto 0);
      |         sm_RFC_IQ_Rx_Buffer_addr  : out std_logic_vector(15-1 downto 0);
      |         sm_RFC_IQ_Rx_Buffer_din   : out std_logic_vector(32-1 downto 0);
      |         sm_RFC_IQ_Rx_Buffer_we    : out std_logic;
      |         -- 'RFB_IQ_Tx_Buffer'
      |         sm_RFB_IQ_Tx_Buffer_dout  : in  std_logic_vector(32-1 downto 0);
      |         sm_RFB_IQ_Tx_Buffer_addr  : out std_logic_vector(15-1 downto 0);
      |         sm_RFB_IQ_Tx_Buffer_din   : out std_logic_vector(32-1 downto 0);
      |         sm_RFB_IQ_Tx_Buffer_we    : out std_logic;
      |         -- 'RFB_RSSI_Buffer'
      |         sm_RFB_RSSI_Buffer_dout  : in  std_logic_vector(32-1 downto 0);
      |         sm_RFB_RSSI_Buffer_addr  : out std_logic_vector(12-1 downto 0);
      |         sm_RFB_RSSI_Buffer_din   : out std_logic_vector(32-1 downto 0);
      |         sm_RFB_RSSI_Buffer_we    : out std_logic;
      |         -- 'RFB_IQ_Rx_Buffer'
      |         sm_RFB_IQ_Rx_Buffer_dout  : in  std_logic_vector(32-1 downto 0);
      |         sm_RFB_IQ_Rx_Buffer_addr  : out std_logic_vector(15-1 downto 0);
      |         sm_RFB_IQ_Rx_Buffer_din   : out std_logic_vector(32-1 downto 0);
      |         sm_RFB_IQ_Rx_Buffer_we    : out std_logic;
      |         -- 'RFA_IQ_Tx_Buffer'
      |         sm_RFA_IQ_Tx_Buffer_dout  : in  std_logic_vector(32-1 downto 0);
      |         sm_RFA_IQ_Tx_Buffer_addr  : out std_logic_vector(15-1 downto 0);
      |         sm_RFA_IQ_Tx_Buffer_din   : out std_logic_vector(32-1 downto 0);
      |         sm_RFA_IQ_Tx_Buffer_we    : out std_logic;
      |         -- 'RFA_RSSI_Buffer'
      |         sm_RFA_RSSI_Buffer_dout  : in  std_logic_vector(32-1 downto 0);
      |         sm_RFA_RSSI_Buffer_addr  : out std_logic_vector(12-1 downto 0);
      |         sm_RFA_RSSI_Buffer_din   : out std_logic_vector(32-1 downto 0);
      |         sm_RFA_RSSI_Buffer_we    : out std_logic;
      |         -- 'RFA_IQ_Rx_Buffer'
      |         sm_RFA_IQ_Rx_Buffer_dout  : in  std_logic_vector(32-1 downto 0);
      |         sm_RFA_IQ_Rx_Buffer_addr  : out std_logic_vector(15-1 downto 0);
      |         sm_RFA_IQ_Rx_Buffer_din   : out std_logic_vector(32-1 downto 0);
      |         sm_RFA_IQ_Rx_Buffer_we    : out std_logic;
      |         shram_en : out std_logic;
      | 
      |         S_AXI_RLAST   : out std_logic;
      |         S_AXI_RID     : out std_logic_vector(C_S_AXI_ID_WIDTH-1 downto 0);
      |         S_AXI_RDATA   : out std_logic_vector(C_S_AXI_DATA_WIDTH-1 downto 0);
      |         S_AXI_RRESP   : out std_logic_vector(1 downto 0);
      |         S_AXI_RVALID  : out std_logic;
      |         S_AXI_RREADY  : in  std_logic
      |     );
      | end entity axi_sgiface;
      | 
      | architecture IMP of axi_sgiface is
      | 
      | -- Internal signals for write channel.
      | signal S_AXI_BVALID_i       : std_logic;
      | signal S_AXI_BID_i          : std_logic_vector(C_S_AXI_ID_WIDTH-1 downto 0);
      | signal S_AXI_WREADY_i       : std_logic;
      |   
      | -- Internal signals for read channels.
      | signal S_AXI_ARLEN_i        : std_logic_vector(C_S_AXI_ARLEN_WIDTH-1 downto 0);
      | signal S_AXI_RLAST_i        : std_logic;
      | signal S_AXI_RREADY_i       : std_logic;
      | signal S_AXI_RVALID_i       : std_logic;
      | signal S_AXI_RDATA_i        : std_logic_vector(C_S_AXI_DATA_WIDTH-1 downto 0);
      | signal S_AXI_RID_i          : std_logic_vector(C_S_AXI_ID_WIDTH-1 downto 0);
      | 
      | -- for read channel
      | signal read_bank_addr_i     : std_logic_vector(C_S_AXI_BANK_ADDR_LEN-1 downto 0);
      | signal read_linear_addr_i   : std_logic_vector(C_S_AXI_LINEAR_ADDR_LEN-1 downto 0);
      | -- for write channel
      | signal write_bank_addr_i    : std_logic_vector(C_S_AXI_BANK_ADDR_LEN-1 downto 0);
      | signal write_linear_addr_i  : std_logic_vector(C_S_AXI_LINEAR_ADDR_LEN-1 downto 0);
      | 
      | signal reg_bank_out_i       : std_logic_vector(C_S_AXI_DATA_WIDTH-1 downto 0);
      | signal fifo_bank_out_i      : std_logic_vector(C_S_AXI_DATA_WIDTH-1 downto 0);
      | signal shmem_bank_out_i     : std_logic_vector(C_S_AXI_DATA_WIDTH-1 downto 0);
      |     
      | -- 'From Register'
      | -- 'BUFF_SIZES'
      | signal sm_BUFF_SIZES_dout_i  : std_logic_vector(C_S_AXI_DATA_WIDTH-1 downto 0);
      | -- 'DESIGN_VER'
      | signal sm_DESIGN_VER_dout_i  : std_logic_vector(C_S_AXI_DATA_WIDTH-1 downto 0);
      | -- 'STATUS'
      | signal sm_STATUS_dout_i  : std_logic_vector(C_S_AXI_DATA_WIDTH-1 downto 0);
      | -- 'RFCD_AGCDoneRSSI'
      | signal sm_RFCD_AGCDoneRSSI_dout_i  : std_logic_vector(C_S_AXI_DATA_WIDTH-1 downto 0);
      | -- 'RFAB_AGCDoneRSSI'
      | signal sm_RFAB_AGCDoneRSSI_dout_i  : std_logic_vector(C_S_AXI_DATA_WIDTH-1 downto 0);
      | -- 'AGCDoneAddr'
      | signal sm_AGCDoneAddr_dout_i  : std_logic_vector(C_S_AXI_DATA_WIDTH-1 downto 0);
      | -- 'To Register'
      | -- 'TxDelay'
      | signal sm_TxDelay_din_i   : std_logic_vector(C_S_AXI_DATA_WIDTH-1 downto 0);
      | signal sm_TxDelay_en_i    : std_logic;
      | signal sm_TxDelay_dout_i  : std_logic_vector(C_S_AXI_DATA_WIDTH-1 downto 0);
      | -- 'RX_BUFF_EN'
      | signal sm_RX_BUFF_EN_din_i   : std_logic_vector(C_S_AXI_DATA_WIDTH-1 downto 0);
      | signal sm_RX_BUFF_EN_en_i    : std_logic;
      | signal sm_RX_BUFF_EN_dout_i  : std_logic_vector(C_S_AXI_DATA_WIDTH-1 downto 0);
      | -- 'CONFIG'
      | signal sm_CONFIG_din_i   : std_logic_vector(C_S_AXI_DATA_WIDTH-1 downto 0);
      | signal sm_CONFIG_en_i    : std_logic;
      | signal sm_CONFIG_dout_i  : std_logic_vector(C_S_AXI_DATA_WIDTH-1 downto 0);
      | -- 'TX_BUFF_EN'
      | signal sm_TX_BUFF_EN_din_i   : std_logic_vector(C_S_AXI_DATA_WIDTH-1 downto 0);
      | signal sm_TX_BUFF_EN_en_i    : std_logic;
      | signal sm_TX_BUFF_EN_dout_i  : std_logic_vector(C_S_AXI_DATA_WIDTH-1 downto 0);
      | -- 'RxLength'
      | signal sm_RxLength_din_i   : std_logic_vector(C_S_AXI_DATA_WIDTH-1 downto 0);
      | signal sm_RxLength_en_i    : std_logic;
      | signal sm_RxLength_dout_i  : std_logic_vector(C_S_AXI_DATA_WIDTH-1 downto 0);
      | -- 'TxLength'
      | signal sm_TxLength_din_i   : std_logic_vector(C_S_AXI_DATA_WIDTH-1 downto 0);
      | signal sm_TxLength_en_i    : std_logic;
      | signal sm_TxLength_dout_i  : std_logic_vector(C_S_AXI_DATA_WIDTH-1 downto 0);
      | -- 'From FIFO'
      | -- 'To FIFO'
      | -- 'Shared Memory'
      | -- 'RFD_IQ_Tx_Buffer'
      | signal sm_RFD_IQ_Tx_Buffer_addr_i  : std_logic_vector(C_S_AXI_LINEAR_ADDR_LEN-1 downto 0);
      | signal sm_RFD_IQ_Tx_Buffer_din_i   : std_logic_vector(C_S_AXI_DATA_WIDTH-1 downto 0);
      | signal sm_RFD_IQ_Tx_Buffer_we_i    : std_logic;
      | signal sm_RFD_IQ_Tx_Buffer_dout_i  : std_logic_vector(C_S_AXI_DATA_WIDTH-1 downto 0);
      | -- 'RFD_RSSI_Buffer'
      | signal sm_RFD_RSSI_Buffer_addr_i  : std_logic_vector(C_S_AXI_LINEAR_ADDR_LEN-1 downto 0);
      | signal sm_RFD_RSSI_Buffer_din_i   : std_logic_vector(C_S_AXI_DATA_WIDTH-1 downto 0);
      | signal sm_RFD_RSSI_Buffer_we_i    : std_logic;
      | signal sm_RFD_RSSI_Buffer_dout_i  : std_logic_vector(C_S_AXI_DATA_WIDTH-1 downto 0);
      | -- 'RFD_IQ_Rx_Buffer'
      | signal sm_RFD_IQ_Rx_Buffer_addr_i  : std_logic_vector(C_S_AXI_LINEAR_ADDR_LEN-1 downto 0);
      | signal sm_RFD_IQ_Rx_Buffer_din_i   : std_logic_vector(C_S_AXI_DATA_WIDTH-1 downto 0);
      | signal sm_RFD_IQ_Rx_Buffer_we_i    : std_logic;
      | signal sm_RFD_IQ_Rx_Buffer_dout_i  : std_logic_vector(C_S_AXI_DATA_WIDTH-1 downto 0);
      | -- 'RFC_IQ_Tx_Buffer'
      | signal sm_RFC_IQ_Tx_Buffer_addr_i  : std_logic_vector(C_S_AXI_LINEAR_ADDR_LEN-1 downto 0);
      | signal sm_RFC_IQ_Tx_Buffer_din_i   : std_logic_vector(C_S_AXI_DATA_WIDTH-1 downto 0);
      | signal sm_RFC_IQ_Tx_Buffer_we_i    : std_logic;
      | signal sm_RFC_IQ_Tx_Buffer_dout_i  : std_logic_vector(C_S_AXI_DATA_WIDTH-1 downto 0);
      | -- 'RFC_RSSI_Buffer'
      | signal sm_RFC_RSSI_Buffer_addr_i  : std_logic_vector(C_S_AXI_LINEAR_ADDR_LEN-1 downto 0);
      | signal sm_RFC_RSSI_Buffer_din_i   : std_logic_vector(C_S_AXI_DATA_WIDTH-1 downto 0);
      | signal sm_RFC_RSSI_Buffer_we_i    : std_logic;
      | signal sm_RFC_RSSI_Buffer_dout_i  : std_logic_vector(C_S_AXI_DATA_WIDTH-1 downto 0);
      | -- 'RFC_IQ_Rx_Buffer'
      | signal sm_RFC_IQ_Rx_Buffer_addr_i  : std_logic_vector(C_S_AXI_LINEAR_ADDR_LEN-1 downto 0);
      | signal sm_RFC_IQ_Rx_Buffer_din_i   : std_logic_vector(C_S_AXI_DATA_WIDTH-1 downto 0);
      | signal sm_RFC_IQ_Rx_Buffer_we_i    : std_logic;
      | signal sm_RFC_IQ_Rx_Buffer_dout_i  : std_logic_vector(C_S_AXI_DATA_WIDTH-1 downto 0);
      | -- 'RFB_IQ_Tx_Buffer'
      | signal sm_RFB_IQ_Tx_Buffer_addr_i  : std_logic_vector(C_S_AXI_LINEAR_ADDR_LEN-1 downto 0);
      | signal sm_RFB_IQ_Tx_Buffer_din_i   : std_logic_vector(C_S_AXI_DATA_WIDTH-1 downto 0);
      | signal sm_RFB_IQ_Tx_Buffer_we_i    : std_logic;
      | signal sm_RFB_IQ_Tx_Buffer_dout_i  : std_logic_vector(C_S_AXI_DATA_WIDTH-1 downto 0);
      | -- 'RFB_RSSI_Buffer'
      | signal sm_RFB_RSSI_Buffer_addr_i  : std_logic_vector(C_S_AXI_LINEAR_ADDR_LEN-1 downto 0);
      | signal sm_RFB_RSSI_Buffer_din_i   : std_logic_vector(C_S_AXI_DATA_WIDTH-1 downto 0);
      | signal sm_RFB_RSSI_Buffer_we_i    : std_logic;
      | signal sm_RFB_RSSI_Buffer_dout_i  : std_logic_vector(C_S_AXI_DATA_WIDTH-1 downto 0);
      | -- 'RFB_IQ_Rx_Buffer'
      | signal sm_RFB_IQ_Rx_Buffer_addr_i  : std_logic_vector(C_S_AXI_LINEAR_ADDR_LEN-1 downto 0);
      | signal sm_RFB_IQ_Rx_Buffer_din_i   : std_logic_vector(C_S_AXI_DATA_WIDTH-1 downto 0);
      | signal sm_RFB_IQ_Rx_Buffer_we_i    : std_logic;
      | signal sm_RFB_IQ_Rx_Buffer_dout_i  : std_logic_vector(C_S_AXI_DATA_WIDTH-1 downto 0);
      | -- 'RFA_IQ_Tx_Buffer'
      | signal sm_RFA_IQ_Tx_Buffer_addr_i  : std_logic_vector(C_S_AXI_LINEAR_ADDR_LEN-1 downto 0);
      | signal sm_RFA_IQ_Tx_Buffer_din_i   : std_logic_vector(C_S_AXI_DATA_WIDTH-1 downto 0);
      | signal sm_RFA_IQ_Tx_Buffer_we_i    : std_logic;
      | signal sm_RFA_IQ_Tx_Buffer_dout_i  : std_logic_vector(C_S_AXI_DATA_WIDTH-1 downto 0);
      | -- 'RFA_RSSI_Buffer'
      | signal sm_RFA_RSSI_Buffer_addr_i  : std_logic_vector(C_S_AXI_LINEAR_ADDR_LEN-1 downto 0);
      | signal sm_RFA_RSSI_Buffer_din_i   : std_logic_vector(C_S_AXI_DATA_WIDTH-1 downto 0);
      | signal sm_RFA_RSSI_Buffer_we_i    : std_logic;
      | signal sm_RFA_RSSI_Buffer_dout_i  : std_logic_vector(C_S_AXI_DATA_WIDTH-1 downto 0);
      | -- 'RFA_IQ_Rx_Buffer'
      | signal sm_RFA_IQ_Rx_Buffer_addr_i  : std_logic_vector(C_S_AXI_LINEAR_ADDR_LEN-1 downto 0);
      | signal sm_RFA_IQ_Rx_Buffer_din_i   : std_logic_vector(C_S_AXI_DATA_WIDTH-1 downto 0);
      | signal sm_RFA_IQ_Rx_Buffer_we_i    : std_logic;
      | signal sm_RFA_IQ_Rx_Buffer_dout_i  : std_logic_vector(C_S_AXI_DATA_WIDTH-1 downto 0);
      | 
      | type t_read_state is (IDLE, READ_PREP, READ_DATA);
      | signal read_state : t_read_state;
      | 
      | type t_write_state is (IDLE, WRITE_DATA, WRITE_RESPONSE);
      | signal write_state : t_write_state;
      | 
      | type t_memmap_state is (READ, WRITE);
      | signal memmap_state : t_memmap_state;
      | 
      | constant C_READ_PREP_DELAY : std_logic_vector(1 downto 0) := "11";
      | 
      | signal read_prep_counter : std_logic_vector(1 downto 0);
      | signal read_addr_counter : std_logic_vector(C_S_AXI_ARLEN_WIDTH-1 downto 0);
      | signal read_data_counter : std_logic_vector(C_S_AXI_ARLEN_WIDTH-1 downto 0);
      | 
      | -- enable of shared BRAMs
      | signal s_shram_en : std_logic;
      | 
      | signal write_addr_valid : std_logic;
      | signal write_ready : std_logic;
      | 
      | -- 're' of From/To FIFOs
      | signal s_fifo_re : std_logic;
      | -- 'we' of To FIFOs
      | signal s_fifo_we : std_logic;
      | 
      | begin
      | 
      | -- enable for 'Shared Memory' blocks
      | shram_en <= s_shram_en;
      | -- RFD_IQ_Tx_Buffer din
      | sm_RFD_IQ_Tx_Buffer_din_i <= S_AXI_WDATA;
      | -- RFD_RSSI_Buffer din
      | sm_RFD_RSSI_Buffer_din_i <= S_AXI_WDATA;
      | -- RFD_IQ_Rx_Buffer din
      | sm_RFD_IQ_Rx_Buffer_din_i <= S_AXI_WDATA;
      | -- RFC_IQ_Tx_Buffer din
      | sm_RFC_IQ_Tx_Buffer_din_i <= S_AXI_WDATA;
      | -- RFC_RSSI_Buffer din
      | sm_RFC_RSSI_Buffer_din_i <= S_AXI_WDATA;
      | -- RFC_IQ_Rx_Buffer din
      | sm_RFC_IQ_Rx_Buffer_din_i <= S_AXI_WDATA;
      | -- RFB_IQ_Tx_Buffer din
      | sm_RFB_IQ_Tx_Buffer_din_i <= S_AXI_WDATA;
      | -- RFB_RSSI_Buffer din
      | sm_RFB_RSSI_Buffer_din_i <= S_AXI_WDATA;
      | -- RFB_IQ_Rx_Buffer din
      | sm_RFB_IQ_Rx_Buffer_din_i <= S_AXI_WDATA;
      | -- RFA_IQ_Tx_Buffer din
      | sm_RFA_IQ_Tx_Buffer_din_i <= S_AXI_WDATA;
      | -- RFA_RSSI_Buffer din
      | sm_RFA_RSSI_Buffer_din_i <= S_AXI_WDATA;
      | -- RFA_IQ_Rx_Buffer din
      | sm_RFA_IQ_Rx_Buffer_din_i <= S_AXI_WDATA;
      | 
      | -- conversion to match with the data bus width
      | -- 'From Register'
      | -- 'BUFF_SIZES'
      | gen_sm_BUFF_SIZES_dout_i: if (32 < C_S_AXI_DATA_WIDTH) generate
      |     sm_BUFF_SIZES_dout_i(C_S_AXI_DATA_WIDTH-1 downto 32) <= (others => '0');
      | end generate gen_sm_BUFF_SIZES_dout_i;
      | sm_BUFF_SIZES_dout_i(32-1 downto 0) <= sm_BUFF_SIZES_dout;
      | -- 'DESIGN_VER'
      | gen_sm_DESIGN_VER_dout_i: if (32 < C_S_AXI_DATA_WIDTH) generate
      |     sm_DESIGN_VER_dout_i(C_S_AXI_DATA_WIDTH-1 downto 32) <= (others => '0');
      | end generate gen_sm_DESIGN_VER_dout_i;
      | sm_DESIGN_VER_dout_i(32-1 downto 0) <= sm_DESIGN_VER_dout;
      | -- 'STATUS'
      | gen_sm_STATUS_dout_i: if (2 < C_S_AXI_DATA_WIDTH) generate
      |     sm_STATUS_dout_i(C_S_AXI_DATA_WIDTH-1 downto 2) <= (others => '0');
      | end generate gen_sm_STATUS_dout_i;
      | sm_STATUS_dout_i(2-1 downto 0) <= sm_STATUS_dout;
      | -- 'RFCD_AGCDoneRSSI'
      | gen_sm_RFCD_AGCDoneRSSI_dout_i: if (32 < C_S_AXI_DATA_WIDTH) generate
      |     sm_RFCD_AGCDoneRSSI_dout_i(C_S_AXI_DATA_WIDTH-1 downto 32) <= (others => '0');
      | end generate gen_sm_RFCD_AGCDoneRSSI_dout_i;
      | sm_RFCD_AGCDoneRSSI_dout_i(32-1 downto 0) <= sm_RFCD_AGCDoneRSSI_dout;
      | -- 'RFAB_AGCDoneRSSI'
      | gen_sm_RFAB_AGCDoneRSSI_dout_i: if (32 < C_S_AXI_DATA_WIDTH) generate
      |     sm_RFAB_AGCDoneRSSI_dout_i(C_S_AXI_DATA_WIDTH-1 downto 32) <= (others => '0');
      | end generate gen_sm_RFAB_AGCDoneRSSI_dout_i;
      | sm_RFAB_AGCDoneRSSI_dout_i(32-1 downto 0) <= sm_RFAB_AGCDoneRSSI_dout;
      | -- 'AGCDoneAddr'
      | gen_sm_AGCDoneAddr_dout_i: if (32 < C_S_AXI_DATA_WIDTH) generate
      |     sm_AGCDoneAddr_dout_i(C_S_AXI_DATA_WIDTH-1 downto 32) <= (others => '0');
      | end generate gen_sm_AGCDoneAddr_dout_i;
      | sm_AGCDoneAddr_dout_i(32-1 downto 0) <= sm_AGCDoneAddr_dout;
      | -- 'To Register'
      | -- 'TxDelay'
      | sm_TxDelay_din     <= sm_TxDelay_din_i(32-1 downto 0);
      | sm_TxDelay_en      <= sm_TxDelay_en_i;
      | gen_sm_TxDelay_dout_i: if (32 < C_S_AXI_DATA_WIDTH) generate
      |     sm_TxDelay_dout_i(C_S_AXI_DATA_WIDTH-1 downto 32) <= (others => '0');
      | end generate gen_sm_TxDelay_dout_i;
      | sm_TxDelay_dout_i(32-1 downto 0) <= sm_TxDelay_dout;
      | -- 'RX_BUFF_EN'
      | sm_RX_BUFF_EN_din     <= sm_RX_BUFF_EN_din_i(32-1 downto 0);
      | sm_RX_BUFF_EN_en      <= sm_RX_BUFF_EN_en_i;
      | gen_sm_RX_BUFF_EN_dout_i: if (32 < C_S_AXI_DATA_WIDTH) generate
      |     sm_RX_BUFF_EN_dout_i(C_S_AXI_DATA_WIDTH-1 downto 32) <= (others => '0');
      | end generate gen_sm_RX_BUFF_EN_dout_i;
      | sm_RX_BUFF_EN_dout_i(32-1 downto 0) <= sm_RX_BUFF_EN_dout;
      | -- 'CONFIG'
      | sm_CONFIG_din     <= sm_CONFIG_din_i(32-1 downto 0);
      | sm_CONFIG_en      <= sm_CONFIG_en_i;
      | gen_sm_CONFIG_dout_i: if (32 < C_S_AXI_DATA_WIDTH) generate
      |     sm_CONFIG_dout_i(C_S_AXI_DATA_WIDTH-1 downto 32) <= (others => '0');
      | end generate gen_sm_CONFIG_dout_i;
      | sm_CONFIG_dout_i(32-1 downto 0) <= sm_CONFIG_dout;
      | -- 'TX_BUFF_EN'
      | sm_TX_BUFF_EN_din     <= sm_TX_BUFF_EN_din_i(32-1 downto 0);
      | sm_TX_BUFF_EN_en      <= sm_TX_BUFF_EN_en_i;
      | gen_sm_TX_BUFF_EN_dout_i: if (32 < C_S_AXI_DATA_WIDTH) generate
      |     sm_TX_BUFF_EN_dout_i(C_S_AXI_DATA_WIDTH-1 downto 32) <= (others => '0');
      | end generate gen_sm_TX_BUFF_EN_dout_i;
      | sm_TX_BUFF_EN_dout_i(32-1 downto 0) <= sm_TX_BUFF_EN_dout;
      | -- 'RxLength'
      | sm_RxLength_din     <= sm_RxLength_din_i(24-1 downto 0);
      | sm_RxLength_en      <= sm_RxLength_en_i;
      | gen_sm_RxLength_dout_i: if (24 < C_S_AXI_DATA_WIDTH) generate
      |     sm_RxLength_dout_i(C_S_AXI_DATA_WIDTH-1 downto 24) <= (others => '0');
      | end generate gen_sm_RxLength_dout_i;
      | sm_RxLength_dout_i(24-1 downto 0) <= sm_RxLength_dout;
      | -- 'TxLength'
      | sm_TxLength_din     <= sm_TxLength_din_i(24-1 downto 0);
      | sm_TxLength_en      <= sm_TxLength_en_i;
      | gen_sm_TxLength_dout_i: if (24 < C_S_AXI_DATA_WIDTH) generate
      |     sm_TxLength_dout_i(C_S_AXI_DATA_WIDTH-1 downto 24) <= (others => '0');
      | end generate gen_sm_TxLength_dout_i;
      | sm_TxLength_dout_i(24-1 downto 0) <= sm_TxLength_dout;
      | -- 'From FIFO'
      | -- 'To FIFO'
      | -- 'Shared Memory'
      | -- 'RFD_IQ_Tx_Buffer'
      | sm_RFD_IQ_Tx_Buffer_addr <= sm_RFD_IQ_Tx_Buffer_addr_i(15-1 downto 0);
      | sm_RFD_IQ_Tx_Buffer_din  <= sm_RFD_IQ_Tx_Buffer_din_i(32-1 downto 0);
      | gen_sm_RFD_IQ_Tx_Buffer_dout_i: if (32 < C_S_AXI_DATA_WIDTH) generate
      |     sm_RFD_IQ_Tx_Buffer_dout_i(C_S_AXI_DATA_WIDTH-1 downto 32) <= (others => '0');
      | end generate gen_sm_RFD_IQ_Tx_Buffer_dout_i;
      | sm_RFD_IQ_Tx_Buffer_dout_i(32-1 downto 0) <= sm_RFD_IQ_Tx_Buffer_dout;
      | sm_RFD_IQ_Tx_Buffer_we <= sm_RFD_IQ_Tx_Buffer_we_i;
      | -- 'RFD_RSSI_Buffer'
      | sm_RFD_RSSI_Buffer_addr <= sm_RFD_RSSI_Buffer_addr_i(12-1 downto 0);
      | sm_RFD_RSSI_Buffer_din  <= sm_RFD_RSSI_Buffer_din_i(32-1 downto 0);
      | gen_sm_RFD_RSSI_Buffer_dout_i: if (32 < C_S_AXI_DATA_WIDTH) generate
      |     sm_RFD_RSSI_Buffer_dout_i(C_S_AXI_DATA_WIDTH-1 downto 32) <= (others => '0');
      | end generate gen_sm_RFD_RSSI_Buffer_dout_i;
      | sm_RFD_RSSI_Buffer_dout_i(32-1 downto 0) <= sm_RFD_RSSI_Buffer_dout;
      | sm_RFD_RSSI_Buffer_we <= sm_RFD_RSSI_Buffer_we_i;
      | -- 'RFD_IQ_Rx_Buffer'
      | sm_RFD_IQ_Rx_Buffer_addr <= sm_RFD_IQ_Rx_Buffer_addr_i(15-1 downto 0);
      | sm_RFD_IQ_Rx_Buffer_din  <= sm_RFD_IQ_Rx_Buffer_din_i(32-1 downto 0);
      | gen_sm_RFD_IQ_Rx_Buffer_dout_i: if (32 < C_S_AXI_DATA_WIDTH) generate
      |     sm_RFD_IQ_Rx_Buffer_dout_i(C_S_AXI_DATA_WIDTH-1 downto 32) <= (others => '0');
      | end generate gen_sm_RFD_IQ_Rx_Buffer_dout_i;
      | sm_RFD_IQ_Rx_Buffer_dout_i(32-1 downto 0) <= sm_RFD_IQ_Rx_Buffer_dout;
      | sm_RFD_IQ_Rx_Buffer_we <= sm_RFD_IQ_Rx_Buffer_we_i;
      | -- 'RFC_IQ_Tx_Buffer'
      | sm_RFC_IQ_Tx_Buffer_addr <= sm_RFC_IQ_Tx_Buffer_addr_i(15-1 downto 0);
      | sm_RFC_IQ_Tx_Buffer_din  <= sm_RFC_IQ_Tx_Buffer_din_i(32-1 downto 0);
      | gen_sm_RFC_IQ_Tx_Buffer_dout_i: if (32 < C_S_AXI_DATA_WIDTH) generate
      |     sm_RFC_IQ_Tx_Buffer_dout_i(C_S_AXI_DATA_WIDTH-1 downto 32) <= (others => '0');
      | end generate gen_sm_RFC_IQ_Tx_Buffer_dout_i;
      | sm_RFC_IQ_Tx_Buffer_dout_i(32-1 downto 0) <= sm_RFC_IQ_Tx_Buffer_dout;
      | sm_RFC_IQ_Tx_Buffer_we <= sm_RFC_IQ_Tx_Buffer_we_i;
      | -- 'RFC_RSSI_Buffer'
      | sm_RFC_RSSI_Buffer_addr <= sm_RFC_RSSI_Buffer_addr_i(12-1 downto 0);
      | sm_RFC_RSSI_Buffer_din  <= sm_RFC_RSSI_Buffer_din_i(32-1 downto 0);
      | gen_sm_RFC_RSSI_Buffer_dout_i: if (32 < C_S_AXI_DATA_WIDTH) generate
      |     sm_RFC_RSSI_Buffer_dout_i(C_S_AXI_DATA_WIDTH-1 downto 32) <= (others => '0');
      | end generate gen_sm_RFC_RSSI_Buffer_dout_i;
      | sm_RFC_RSSI_Buffer_dout_i(32-1 downto 0) <= sm_RFC_RSSI_Buffer_dout;
      | sm_RFC_RSSI_Buffer_we <= sm_RFC_RSSI_Buffer_we_i;
      | -- 'RFC_IQ_Rx_Buffer'
      | sm_RFC_IQ_Rx_Buffer_addr <= sm_RFC_IQ_Rx_Buffer_addr_i(15-1 downto 0);
      | sm_RFC_IQ_Rx_Buffer_din  <= sm_RFC_IQ_Rx_Buffer_din_i(32-1 downto 0);
      | gen_sm_RFC_IQ_Rx_Buffer_dout_i: if (32 < C_S_AXI_DATA_WIDTH) generate
      |     sm_RFC_IQ_Rx_Buffer_dout_i(C_S_AXI_DATA_WIDTH-1 downto 32) <= (others => '0');
      | end generate gen_sm_RFC_IQ_Rx_Buffer_dout_i;
      | sm_RFC_IQ_Rx_Buffer_dout_i(32-1 downto 0) <= sm_RFC_IQ_Rx_Buffer_dout;
      | sm_RFC_IQ_Rx_Buffer_we <= sm_RFC_IQ_Rx_Buffer_we_i;
      | -- 'RFB_IQ_Tx_Buffer'
      | sm_RFB_IQ_Tx_Buffer_addr <= sm_RFB_IQ_Tx_Buffer_addr_i(15-1 downto 0);
      | sm_RFB_IQ_Tx_Buffer_din  <= sm_RFB_IQ_Tx_Buffer_din_i(32-1 downto 0);
      | gen_sm_RFB_IQ_Tx_Buffer_dout_i: if (32 < C_S_AXI_DATA_WIDTH) generate
      |     sm_RFB_IQ_Tx_Buffer_dout_i(C_S_AXI_DATA_WIDTH-1 downto 32) <= (others => '0');
      | end generate gen_sm_RFB_IQ_Tx_Buffer_dout_i;
      | sm_RFB_IQ_Tx_Buffer_dout_i(32-1 downto 0) <= sm_RFB_IQ_Tx_Buffer_dout;
      | sm_RFB_IQ_Tx_Buffer_we <= sm_RFB_IQ_Tx_Buffer_we_i;
      | -- 'RFB_RSSI_Buffer'
      | sm_RFB_RSSI_Buffer_addr <= sm_RFB_RSSI_Buffer_addr_i(12-1 downto 0);
      | sm_RFB_RSSI_Buffer_din  <= sm_RFB_RSSI_Buffer_din_i(32-1 downto 0);
      | gen_sm_RFB_RSSI_Buffer_dout_i: if (32 < C_S_AXI_DATA_WIDTH) generate
      |     sm_RFB_RSSI_Buffer_dout_i(C_S_AXI_DATA_WIDTH-1 downto 32) <= (others => '0');
      | end generate gen_sm_RFB_RSSI_Buffer_dout_i;
      | sm_RFB_RSSI_Buffer_dout_i(32-1 downto 0) <= sm_RFB_RSSI_Buffer_dout;
      | sm_RFB_RSSI_Buffer_we <= sm_RFB_RSSI_Buffer_we_i;
      | -- 'RFB_IQ_Rx_Buffer'
      | sm_RFB_IQ_Rx_Buffer_addr <= sm_RFB_IQ_Rx_Buffer_addr_i(15-1 downto 0);
      | sm_RFB_IQ_Rx_Buffer_din  <= sm_RFB_IQ_Rx_Buffer_din_i(32-1 downto 0);
      | gen_sm_RFB_IQ_Rx_Buffer_dout_i: if (32 < C_S_AXI_DATA_WIDTH) generate
      |     sm_RFB_IQ_Rx_Buffer_dout_i(C_S_AXI_DATA_WIDTH-1 downto 32) <= (others => '0');
      | end generate gen_sm_RFB_IQ_Rx_Buffer_dout_i;
      | sm_RFB_IQ_Rx_Buffer_dout_i(32-1 downto 0) <= sm_RFB_IQ_Rx_Buffer_dout;
      | sm_RFB_IQ_Rx_Buffer_we <= sm_RFB_IQ_Rx_Buffer_we_i;
      | -- 'RFA_IQ_Tx_Buffer'
      | sm_RFA_IQ_Tx_Buffer_addr <= sm_RFA_IQ_Tx_Buffer_addr_i(15-1 downto 0);
      | sm_RFA_IQ_Tx_Buffer_din  <= sm_RFA_IQ_Tx_Buffer_din_i(32-1 downto 0);
      | gen_sm_RFA_IQ_Tx_Buffer_dout_i: if (32 < C_S_AXI_DATA_WIDTH) generate
      |     sm_RFA_IQ_Tx_Buffer_dout_i(C_S_AXI_DATA_WIDTH-1 downto 32) <= (others => '0');
      | end generate gen_sm_RFA_IQ_Tx_Buffer_dout_i;
      | sm_RFA_IQ_Tx_Buffer_dout_i(32-1 downto 0) <= sm_RFA_IQ_Tx_Buffer_dout;
      | sm_RFA_IQ_Tx_Buffer_we <= sm_RFA_IQ_Tx_Buffer_we_i;
      | -- 'RFA_RSSI_Buffer'
      | sm_RFA_RSSI_Buffer_addr <= sm_RFA_RSSI_Buffer_addr_i(12-1 downto 0);
      | sm_RFA_RSSI_Buffer_din  <= sm_RFA_RSSI_Buffer_din_i(32-1 downto 0);
      | gen_sm_RFA_RSSI_Buffer_dout_i: if (32 < C_S_AXI_DATA_WIDTH) generate
      |     sm_RFA_RSSI_Buffer_dout_i(C_S_AXI_DATA_WIDTH-1 downto 32) <= (others => '0');
      | end generate gen_sm_RFA_RSSI_Buffer_dout_i;
      | sm_RFA_RSSI_Buffer_dout_i(32-1 downto 0) <= sm_RFA_RSSI_Buffer_dout;
      | sm_RFA_RSSI_Buffer_we <= sm_RFA_RSSI_Buffer_we_i;
      | -- 'RFA_IQ_Rx_Buffer'
      | sm_RFA_IQ_Rx_Buffer_addr <= sm_RFA_IQ_Rx_Buffer_addr_i(15-1 downto 0);
      | sm_RFA_IQ_Rx_Buffer_din  <= sm_RFA_IQ_Rx_Buffer_din_i(32-1 downto 0);
      | gen_sm_RFA_IQ_Rx_Buffer_dout_i: if (32 < C_S_AXI_DATA_WIDTH) generate
      |     sm_RFA_IQ_Rx_Buffer_dout_i(C_S_AXI_DATA_WIDTH-1 downto 32) <= (others => '0');
      | end generate gen_sm_RFA_IQ_Rx_Buffer_dout_i;
      | sm_RFA_IQ_Rx_Buffer_dout_i(32-1 downto 0) <= sm_RFA_IQ_Rx_Buffer_dout;
      | sm_RFA_IQ_Rx_Buffer_we <= sm_RFA_IQ_Rx_Buffer_we_i;
      | 
      | ReadWriteSelect: process(memmap_state) is begin
      |     if (memmap_state = READ) then
      |         -- 'RFD_IQ_Tx_Buffer'
      |         sm_RFD_IQ_Tx_Buffer_addr_i <= read_linear_addr_i;-- 'RFD_RSSI_Buffer'
      |         sm_RFD_RSSI_Buffer_addr_i <= read_linear_addr_i;-- 'RFD_IQ_Rx_Buffer'
      |         sm_RFD_IQ_Rx_Buffer_addr_i <= read_linear_addr_i;-- 'RFC_IQ_Tx_Buffer'
      |         sm_RFC_IQ_Tx_Buffer_addr_i <= read_linear_addr_i;-- 'RFC_RSSI_Buffer'
      |         sm_RFC_RSSI_Buffer_addr_i <= read_linear_addr_i;-- 'RFC_IQ_Rx_Buffer'
      |         sm_RFC_IQ_Rx_Buffer_addr_i <= read_linear_addr_i;-- 'RFB_IQ_Tx_Buffer'
      |         sm_RFB_IQ_Tx_Buffer_addr_i <= read_linear_addr_i;-- 'RFB_RSSI_Buffer'
      |         sm_RFB_RSSI_Buffer_addr_i <= read_linear_addr_i;-- 'RFB_IQ_Rx_Buffer'
      |         sm_RFB_IQ_Rx_Buffer_addr_i <= read_linear_addr_i;-- 'RFA_IQ_Tx_Buffer'
      |         sm_RFA_IQ_Tx_Buffer_addr_i <= read_linear_addr_i;-- 'RFA_RSSI_Buffer'
      |         sm_RFA_RSSI_Buffer_addr_i <= read_linear_addr_i;-- 'RFA_IQ_Rx_Buffer'
      |         sm_RFA_IQ_Rx_Buffer_addr_i <= read_linear_addr_i;
      |     else
      |         -- 'RFD_IQ_Tx_Buffer'
      |         sm_RFD_IQ_Tx_Buffer_addr_i <= write_linear_addr_i;-- 'RFD_RSSI_Buffer'
      |         sm_RFD_RSSI_Buffer_addr_i <= write_linear_addr_i;-- 'RFD_IQ_Rx_Buffer'
      |         sm_RFD_IQ_Rx_Buffer_addr_i <= write_linear_addr_i;-- 'RFC_IQ_Tx_Buffer'
      |         sm_RFC_IQ_Tx_Buffer_addr_i <= write_linear_addr_i;-- 'RFC_RSSI_Buffer'
      |         sm_RFC_RSSI_Buffer_addr_i <= write_linear_addr_i;-- 'RFC_IQ_Rx_Buffer'
      |         sm_RFC_IQ_Rx_Buffer_addr_i <= write_linear_addr_i;-- 'RFB_IQ_Tx_Buffer'
      |         sm_RFB_IQ_Tx_Buffer_addr_i <= write_linear_addr_i;-- 'RFB_RSSI_Buffer'
      |         sm_RFB_RSSI_Buffer_addr_i <= write_linear_addr_i;-- 'RFB_IQ_Rx_Buffer'
      |         sm_RFB_IQ_Rx_Buffer_addr_i <= write_linear_addr_i;-- 'RFA_IQ_Tx_Buffer'
      |         sm_RFA_IQ_Tx_Buffer_addr_i <= write_linear_addr_i;-- 'RFA_RSSI_Buffer'
      |         sm_RFA_RSSI_Buffer_addr_i <= write_linear_addr_i;-- 'RFA_IQ_Rx_Buffer'
      |         sm_RFA_IQ_Rx_Buffer_addr_i <= write_linear_addr_i;
      |     end if;
      | end process ReadWriteSelect;
      | 
      | -----------------------------------------------------------------------------
      | -- address for 'Shared Memory'
      | -----------------------------------------------------------------------------
      | SharedMemory_Addr_ResetN : process(AXI_AClk) is begin
      |     if (AXI_AClk'event and AXI_AClk = '1') then
      |         if (AXI_AResetN = '0') then
      |             memmap_state <= READ;
      |         else
      |             if (S_AXI_AWVALID = '1') then
      |                 -- write operation
      |                 memmap_state <= WRITE;
      |             elsif (S_AXI_ARVALID = '1') then
      |                 -- read operation
      |                 memmap_state <= READ;
      |             end if;
      |         end if;
      |     end if;
      | end process SharedMemory_Addr_ResetN;
      | 
      | -----------------------------------------------------------------------------
      | -- WRITE Command Control
      | -----------------------------------------------------------------------------
      | S_AXI_BID     <= S_AXI_BID_i;
      | S_AXI_BVALID  <= S_AXI_BVALID_i;
      | S_AXI_WREADY  <= S_AXI_WREADY_i;
      | -- No error checking
      | S_AXI_BRESP  <= (others=>'0');
      | 
      | PROC_AWREADY_ACK: process(read_state, write_state, S_AXI_ARVALID, S_AXI_AWVALID) is begin
      |     if (write_state = IDLE and S_AXI_AWVALID = '1' and read_state = IDLE) then
      |         S_AXI_AWREADY <= S_AXI_AWVALID;
      |     else
      |         S_AXI_AWREADY <= '0';
      |     end if;
      | end process PROC_AWREADY_ACK;
      | 
      | Cmd_Decode_Write: process(AXI_AClk) is begin
      |     if (AXI_AClk'event and AXI_AClk = '1') then
      |         if (AXI_AResetN = '0') then
      |             write_addr_valid    <= '0';
      |             write_ready         <= '0';
      |             s_fifo_we           <= '0';
      |             S_AXI_BVALID_i      <= '0';
      |             S_AXI_BID_i         <= (others => '0');
      |             write_bank_addr_i   <= (others => '0');
      |             write_linear_addr_i <= (others => '0');
      |         else
      |             if (write_state = IDLE) then
      |                 if (S_AXI_AWVALID = '1' and read_state = IDLE) then
      |                     -- reflect awid
      |                     S_AXI_BID_i <= S_AXI_AWID;
      | 
      |                     -- latch bank and linear addresses
      |                     write_bank_addr_i   <= S_AXI_AWADDR(C_S_AXI_TOTAL_ADDR_LEN-1 downto C_S_AXI_LINEAR_ADDR_LEN+2);
      |                     write_linear_addr_i <= S_AXI_AWADDR(C_S_AXI_LINEAR_ADDR_LEN+1 downto 2);
      |                     write_addr_valid <= '1';
      |                     s_fifo_we <= '1';
      | 
      |                     -- write state transition
      |                     write_state <= WRITE_DATA;
      |                 end if;
      |             elsif (write_state = WRITE_DATA) then
      |                 write_ready <= '1';
      |                 s_fifo_we <= '0';
      |                 write_addr_valid <= S_AXI_WVALID;
      |                 
      |                 if (S_AXI_WVALID = '1' and write_ready = '1') then
      |                     write_linear_addr_i <= Std_Logic_Vector(unsigned(write_linear_addr_i) + 1);
      |                 end if;
      | 
      |                 if (S_AXI_WLAST = '1' and write_ready = '1') then
      |                     -- start responding through B channel upon the last write data sample
      |                     S_AXI_BVALID_i <= '1';
      |                     -- write data is over
      |                     write_addr_valid <= '0';
      |                     write_ready <= '0';
      |                     -- write state transition
      |                     write_state <= WRITE_RESPONSE;
      |                 end if;
      |             elsif (write_state = WRITE_RESPONSE) then
      | 
      |                 if (S_AXI_BREADY = '1') then
      |                     -- write respond is over
      |                     S_AXI_BVALID_i <= '0';
      |                     S_AXI_BID_i <= (others => '0');
      | 
      |                     -- write state transition
      |                     write_state <= IDLE;
      |                 end if;
      |             end if;
      |         end if;
      |     end if;
      | end process Cmd_Decode_Write;
      | 
      | Write_Linear_Addr_Decode : process(AXI_AClk) is 
      | 
      | begin
      |     if (AXI_AClk'event and AXI_AClk = '1') then
      |         if (AXI_AResetN = '0') then
      |             -- 'To Register'
      |             -- TxDelay din/en
      |             sm_TxDelay_din_i <= (others => '0');
      |             sm_TxDelay_en_i <= '0';
      |             -- RX_BUFF_EN din/en
      |             sm_RX_BUFF_EN_din_i <= (others => '0');
      |             sm_RX_BUFF_EN_en_i <= '0';
      |             -- CONFIG din/en
      |             sm_CONFIG_din_i <= (others => '0');
      |             sm_CONFIG_en_i <= '0';
      |             -- TX_BUFF_EN din/en
      |             sm_TX_BUFF_EN_din_i <= (others => '0');
      |             sm_TX_BUFF_EN_en_i <= '0';
      |             -- RxLength din/en
      |             sm_RxLength_din_i <= (others => '0');
      |             sm_RxLength_en_i <= '0';
      |             -- TxLength din/en
      |             sm_TxLength_din_i <= (others => '0');
      |             sm_TxLength_en_i <= '0';
      |             -- 'To FIFO'
      |             -- 'Shared Memory'
      |             -- RFD_IQ_Tx_Buffer we
      |             sm_RFD_IQ_Tx_Buffer_we_i <= '0';
      |             -- RFD_RSSI_Buffer we
      |             sm_RFD_RSSI_Buffer_we_i <= '0';
      |             -- RFD_IQ_Rx_Buffer we
      |             sm_RFD_IQ_Rx_Buffer_we_i <= '0';
      |             -- RFC_IQ_Tx_Buffer we
      |             sm_RFC_IQ_Tx_Buffer_we_i <= '0';
      |             -- RFC_RSSI_Buffer we
      |             sm_RFC_RSSI_Buffer_we_i <= '0';
      |             -- RFC_IQ_Rx_Buffer we
      |             sm_RFC_IQ_Rx_Buffer_we_i <= '0';
      |             -- RFB_IQ_Tx_Buffer we
      |             sm_RFB_IQ_Tx_Buffer_we_i <= '0';
      |             -- RFB_RSSI_Buffer we
      |             sm_RFB_RSSI_Buffer_we_i <= '0';
      |             -- RFB_IQ_Rx_Buffer we
      |             sm_RFB_IQ_Rx_Buffer_we_i <= '0';
      |             -- RFA_IQ_Tx_Buffer we
      |             sm_RFA_IQ_Tx_Buffer_we_i <= '0';
      |             -- RFA_RSSI_Buffer we
      |             sm_RFA_RSSI_Buffer_we_i <= '0';
      |             -- RFA_IQ_Rx_Buffer we
      |             sm_RFA_IQ_Rx_Buffer_we_i <= '0';
      |         else
      |             -- default assignments
      |             -- RFD_IQ_Tx_Buffer we
      |             sm_RFD_IQ_Tx_Buffer_we_i <= '0';
      |             -- RFD_RSSI_Buffer we
      |             sm_RFD_RSSI_Buffer_we_i <= '0';
      |             -- RFD_IQ_Rx_Buffer we
      |             sm_RFD_IQ_Rx_Buffer_we_i <= '0';
      |             -- RFC_IQ_Tx_Buffer we
      |             sm_RFC_IQ_Tx_Buffer_we_i <= '0';
      |             -- RFC_RSSI_Buffer we
      |             sm_RFC_RSSI_Buffer_we_i <= '0';
      |             -- RFC_IQ_Rx_Buffer we
      |             sm_RFC_IQ_Rx_Buffer_we_i <= '0';
      |             -- RFB_IQ_Tx_Buffer we
      |             sm_RFB_IQ_Tx_Buffer_we_i <= '0';
      |             -- RFB_RSSI_Buffer we
      |             sm_RFB_RSSI_Buffer_we_i <= '0';
      |             -- RFB_IQ_Rx_Buffer we
      |             sm_RFB_IQ_Rx_Buffer_we_i <= '0';
      |             -- RFA_IQ_Tx_Buffer we
      |             sm_RFA_IQ_Tx_Buffer_we_i <= '0';
      |             -- RFA_RSSI_Buffer we
      |             sm_RFA_RSSI_Buffer_we_i <= '0';
      |             -- RFA_IQ_Rx_Buffer we
      |             sm_RFA_IQ_Rx_Buffer_we_i <= '0';
      | 
      |             -- 'To Register'
      |             if (unsigned(write_bank_addr_i) = 2) then
      |                 if (unsigned(write_linear_addr_i) = 0) then
      |                     -- TxDelay din/en
      |                     sm_TxDelay_din_i <= S_AXI_WDATA;
      |                     sm_TxDelay_en_i  <= write_addr_valid;
      |                 elsif (unsigned(write_linear_addr_i) = 1) then
      |                     -- RX_BUFF_EN din/en
      |                     sm_RX_BUFF_EN_din_i <= S_AXI_WDATA;
      |                     sm_RX_BUFF_EN_en_i  <= write_addr_valid;
      |                 elsif (unsigned(write_linear_addr_i) = 2) then
      |                     -- CONFIG din/en
      |                     sm_CONFIG_din_i <= S_AXI_WDATA;
      |                     sm_CONFIG_en_i  <= write_addr_valid;
      |                 elsif (unsigned(write_linear_addr_i) = 3) then
      |                     -- TX_BUFF_EN din/en
      |                     sm_TX_BUFF_EN_din_i <= S_AXI_WDATA;
      |                     sm_TX_BUFF_EN_en_i  <= write_addr_valid;
      |                 elsif (unsigned(write_linear_addr_i) = 4) then
      |                     -- RxLength din/en
      |                     sm_RxLength_din_i <= S_AXI_WDATA;
      |                     sm_RxLength_en_i  <= write_addr_valid;
      |                 elsif (unsigned(write_linear_addr_i) = 5) then
      |                     -- TxLength din/en
      |                     sm_TxLength_din_i <= S_AXI_WDATA;
      |                     sm_TxLength_en_i  <= write_addr_valid;
      |                 end if;
      |             end if;        
      |         
      |             -- 'Shared Memory'
      |             if unsigned(write_bank_addr_i) = 0 then
      |                 if (unsigned(write_linear_addr_i(C_S_AXI_LINEAR_ADDR_LEN-1 downto 15)) = 0) then
      |                     -- RFD_IQ_Tx_Buffer we
      |                     sm_RFD_IQ_Tx_Buffer_we_i  <= write_addr_valid;
      |                 elsif (unsigned(write_linear_addr_i(C_S_AXI_LINEAR_ADDR_LEN-1 downto 12)) = 64) then
      |                     -- RFD_RSSI_Buffer we
      |                     sm_RFD_RSSI_Buffer_we_i  <= write_addr_valid;
      |                 elsif (unsigned(write_linear_addr_i(C_S_AXI_LINEAR_ADDR_LEN-1 downto 15)) = 1) then
      |                     -- RFD_IQ_Rx_Buffer we
      |                     sm_RFD_IQ_Rx_Buffer_we_i  <= write_addr_valid;
      |                 elsif (unsigned(write_linear_addr_i(C_S_AXI_LINEAR_ADDR_LEN-1 downto 15)) = 2) then
      |                     -- RFC_IQ_Tx_Buffer we
      |                     sm_RFC_IQ_Tx_Buffer_we_i  <= write_addr_valid;
      |                 elsif (unsigned(write_linear_addr_i(C_S_AXI_LINEAR_ADDR_LEN-1 downto 12)) = 65) then
      |                     -- RFC_RSSI_Buffer we
      |                     sm_RFC_RSSI_Buffer_we_i  <= write_addr_valid;
      |                 elsif (unsigned(write_linear_addr_i(C_S_AXI_LINEAR_ADDR_LEN-1 downto 15)) = 3) then
      |                     -- RFC_IQ_Rx_Buffer we
      |                     sm_RFC_IQ_Rx_Buffer_we_i  <= write_addr_valid;
      |                 elsif (unsigned(write_linear_addr_i(C_S_AXI_LINEAR_ADDR_LEN-1 downto 15)) = 4) then
      |                     -- RFB_IQ_Tx_Buffer we
      |                     sm_RFB_IQ_Tx_Buffer_we_i  <= write_addr_valid;
      |                 elsif (unsigned(write_linear_addr_i(C_S_AXI_LINEAR_ADDR_LEN-1 downto 12)) = 66) then
      |                     -- RFB_RSSI_Buffer we
      |                     sm_RFB_RSSI_Buffer_we_i  <= write_addr_valid;
      |                 elsif (unsigned(write_linear_addr_i(C_S_AXI_LINEAR_ADDR_LEN-1 downto 15)) = 5) then
      |                     -- RFB_IQ_Rx_Buffer we
      |                     sm_RFB_IQ_Rx_Buffer_we_i  <= write_addr_valid;
      |                 elsif (unsigned(write_linear_addr_i(C_S_AXI_LINEAR_ADDR_LEN-1 downto 15)) = 6) then
      |                     -- RFA_IQ_Tx_Buffer we
      |                     sm_RFA_IQ_Tx_Buffer_we_i  <= write_addr_valid;
      |                 elsif (unsigned(write_linear_addr_i(C_S_AXI_LINEAR_ADDR_LEN-1 downto 12)) = 67) then
      |                     -- RFA_RSSI_Buffer we
      |                     sm_RFA_RSSI_Buffer_we_i  <= write_addr_valid;
      |                 elsif (unsigned(write_linear_addr_i(C_S_AXI_LINEAR_ADDR_LEN-1 downto 15)) = 7) then
      |                     -- RFA_IQ_Rx_Buffer we
      |                     sm_RFA_IQ_Rx_Buffer_we_i  <= write_addr_valid;
      |                 end if;
      |             end if;        
      |         end if;
      |     end if;
      | end process Write_Linear_Addr_Decode;
      |  
      | -----------------------------------------------------------------------------
      | -- READ Control
      | -----------------------------------------------------------------------------
      | 
      | S_AXI_RDATA  <= S_AXI_RDATA_i;
      | S_AXI_RVALID  <= S_AXI_RVALID_i;
      | S_AXI_RLAST   <= S_AXI_RLAST_i;
      | S_AXI_RID     <= S_AXI_RID_i;
      | -- TODO: no error checking
      | S_AXI_RRESP <= (others=>'0');
      | 
      | PROC_ARREADY_ACK: process(read_state, S_AXI_ARVALID, write_state, S_AXI_AWVALID) is begin
      |     -- Note: WRITE has higher priority than READ
      |     if (read_state = IDLE and S_AXI_ARVALID = '1' and write_state = IDLE and S_AXI_AWVALID /= '1') then
      |         S_AXI_ARREADY <= S_AXI_ARVALID;
      |     else
      |         S_AXI_ARREADY <= '0';
      |     end if;
      | end process PROC_ARREADY_ACK;
      | 
      | S_AXI_WREADY_i <= write_ready;
      | 
      | Process_Sideband: process(write_state, read_state) is begin
      |     if (read_state = READ_PREP) then
      |         s_shram_en <= '1';
      |     elsif (read_state = READ_DATA) then
      |         s_shram_en <= S_AXI_RREADY;
      |     elsif (write_state = WRITE_DATA) then
      |         s_shram_en <= S_AXI_WVALID;
      |     else
      |         s_shram_en <= '0';
      |     end if;
      | end process Process_Sideband;
      | 
      | Cmd_Decode_Read: process(AXI_AClk) is begin
      |     if (AXI_AClk'event and AXI_AClk = '1') then
      |         if (AXI_AResetN = '0') then
      |             S_AXI_RVALID_i <= '0';
      |             read_bank_addr_i    <= (others => '0');
      |             read_linear_addr_i  <= (others => '0');
      |             S_AXI_ARLEN_i       <= (others => '0');
      |             S_AXI_RLAST_i       <= '0';
      |             S_AXI_RID_i         <= (others => '0');
      |             read_state          <= IDLE;
      |             read_prep_counter   <= (others => '0');
      |             read_addr_counter   <= (others => '0');
      |             read_data_counter   <= (others => '0');
      |         else
      |             -- default assignments
      |             s_fifo_re <= '0';
      | 
      |             if (read_state = IDLE) then
      |                 -- Note WRITE has higher priority than READ
      |                 if (S_AXI_ARVALID = '1' and write_state = IDLE and S_AXI_AWVALID /= '1') then
      |                     -- extract bank and linear addresses
      |                     read_bank_addr_i    <= S_AXI_ARADDR(C_S_AXI_TOTAL_ADDR_LEN-1 downto C_S_AXI_LINEAR_ADDR_LEN+2);
      |                     read_linear_addr_i  <= S_AXI_ARADDR(C_S_AXI_LINEAR_ADDR_LEN+1 downto 2);
      |                     s_fifo_re <= '1';
      | 
      |                     -- reflect arid
      |                     S_AXI_RID_i <= S_AXI_ARID;
      | 
      |                     -- load read liner address and data counter
      |                     read_addr_counter <= S_AXI_ARLEN;
      |                     read_data_counter <= S_AXI_ARLEN;
      | 
      |                     -- load read preparation counter
      |                     read_prep_counter <= C_READ_PREP_DELAY;
      |                     -- read state transition
      |                     read_state <= READ_PREP;
      |                 end if;
      |             elsif (read_state = READ_PREP) then
      |                 if (unsigned(read_prep_counter) = 0) then
      |                     if (unsigned(read_data_counter) = 0) then
      |                         -- tag the last data generated by the slave
      |                         S_AXI_RLAST_i <= '1';
      |                     end if;
      |                     -- valid data appears
      |                     S_AXI_RVALID_i <= '1';
      |                     -- read state transition
      |                     read_state <= READ_DATA;
      |                 else
      |                     -- decrease read preparation counter
      |                     read_prep_counter <= Std_Logic_Vector(unsigned(read_prep_counter) - 1);
      |                 end if;
      | 
      |                 if (unsigned(read_prep_counter) /= 3 and unsigned(read_addr_counter) /= 0) then
      |                     -- decrease address counter
      |                     read_addr_counter <= Std_Logic_Vector(unsigned(read_addr_counter) - 1);
      |                     -- increase linear address (no band crossing)
      |                     read_linear_addr_i <= Std_Logic_Vector(unsigned(read_linear_addr_i) + 1);
      |                 end if;
      |             elsif (read_state = READ_DATA) then
      |                 if (S_AXI_RREADY = '1') then
      |                     if (unsigned(read_data_counter) = 1) then
      |                         -- tag the last data generated by the slave
      |                         S_AXI_RLAST_i <= '1';
      |                     end if;
      | 
      |                     if (unsigned(read_data_counter) = 0) then
      |                         -- arid
      |                         S_AXI_RID_i <= (others => '0');
      |                         -- rlast
      |                         S_AXI_RLAST_i <= '0';
      |                         -- no more valid data
      |                         S_AXI_RVALID_i <= '0';
      |                         -- read state transition
      |                         read_state <= IDLE;
      |                     else
      |                         -- decrease read preparation counter
      |                         read_data_counter <= Std_Logic_Vector(unsigned(read_data_counter) - 1);
      | 
      |                         if (unsigned(read_addr_counter) /= 0) then
      |                             -- decrease address counter
      |                             read_addr_counter <= Std_Logic_Vector(unsigned(read_addr_counter) - 1);
      |                             -- increase linear address (no band crossing)
      |                             read_linear_addr_i <= Std_Logic_Vector(unsigned(read_linear_addr_i) + 1);
      |                         end if;
      |                     end if;
      |                 end if;
      |             end if;
      | 
      |         end if;
      |     end if;
      | end process Cmd_Decode_Read;
      | 
      | Read_Linear_Addr_Decode : process(AXI_AClk) is begin
      |     if (AXI_AClk'event and AXI_AClk = '1') then
      |         if (AXI_AResetN = '0') then
      |             reg_bank_out_i   <= (others => '0');
      |             fifo_bank_out_i  <= (others => '0');
      |             shmem_bank_out_i <= (others => '0');
      |             S_AXI_RDATA_i    <= (others => '0');
      |         else
      |             if (unsigned(read_bank_addr_i) = 2) then
      |                 -- 'From Register'
      |                 if (unsigned(read_linear_addr_i) = 6) then
      |                     -- 'BUFF_SIZES' dout
      |                     reg_bank_out_i <= sm_BUFF_SIZES_dout_i;
      |                 elsif (unsigned(read_linear_addr_i) = 7) then
      |                     -- 'DESIGN_VER' dout
      |                     reg_bank_out_i <= sm_DESIGN_VER_dout_i;
      |                 elsif (unsigned(read_linear_addr_i) = 8) then
      |                     -- 'STATUS' dout
      |                     reg_bank_out_i <= sm_STATUS_dout_i;
      |                 elsif (unsigned(read_linear_addr_i) = 9) then
      |                     -- 'RFCD_AGCDoneRSSI' dout
      |                     reg_bank_out_i <= sm_RFCD_AGCDoneRSSI_dout_i;
      |                 elsif (unsigned(read_linear_addr_i) = 10) then
      |                     -- 'RFAB_AGCDoneRSSI' dout
      |                     reg_bank_out_i <= sm_RFAB_AGCDoneRSSI_dout_i;
      |                 elsif (unsigned(read_linear_addr_i) = 11) then
      |                     -- 'AGCDoneAddr' dout
      |                     reg_bank_out_i <= sm_AGCDoneAddr_dout_i;
      |                 end if;
      |                 -- 'To Register' (with register readback)
      |                 if (unsigned(read_linear_addr_i) = 0) then
      |                     -- 'TxDelay' dout
      |                     reg_bank_out_i <= sm_TxDelay_dout_i;
      |                 elsif (unsigned(read_linear_addr_i) = 1) then
      |                     -- 'RX_BUFF_EN' dout
      |                     reg_bank_out_i <= sm_RX_BUFF_EN_dout_i;
      |                 elsif (unsigned(read_linear_addr_i) = 2) then
      |                     -- 'CONFIG' dout
      |                     reg_bank_out_i <= sm_CONFIG_dout_i;
      |                 elsif (unsigned(read_linear_addr_i) = 3) then
      |                     -- 'TX_BUFF_EN' dout
      |                     reg_bank_out_i <= sm_TX_BUFF_EN_dout_i;
      |                 elsif (unsigned(read_linear_addr_i) = 4) then
      |                     -- 'RxLength' dout
      |                     reg_bank_out_i <= sm_RxLength_dout_i;
      |                 elsif (unsigned(read_linear_addr_i) = 5) then
      |                     -- 'TxLength' dout
      |                     reg_bank_out_i <= sm_TxLength_dout_i;
      |                 end if;
      | 
      |                 S_AXI_RDATA_i <= reg_bank_out_i;
      |             elsif (unsigned(read_bank_addr_i) = 1) then
      |                 -- 'From FIFO'
      |                 -- 'To FIFO'
      | 
      |                 S_AXI_RDATA_i <= fifo_bank_out_i;
      |             elsif (unsigned(read_bank_addr_i) = 0 and s_shram_en = '1') then
      |                 -- 'Shared Memory'
      |                 if (unsigned(read_linear_addr_i(C_S_AXI_LINEAR_ADDR_LEN-1 downto 15)) = 0) then
      |                     -- 'RFD_IQ_Tx_Buffer' dout
      |                     shmem_bank_out_i <= sm_RFD_IQ_Tx_Buffer_dout_i;
      |                 elsif (unsigned(read_linear_addr_i(C_S_AXI_LINEAR_ADDR_LEN-1 downto 12)) = 64) then
      |                     -- 'RFD_RSSI_Buffer' dout
      |                     shmem_bank_out_i <= sm_RFD_RSSI_Buffer_dout_i;
      |                 elsif (unsigned(read_linear_addr_i(C_S_AXI_LINEAR_ADDR_LEN-1 downto 15)) = 1) then
      |                     -- 'RFD_IQ_Rx_Buffer' dout
      |                     shmem_bank_out_i <= sm_RFD_IQ_Rx_Buffer_dout_i;
      |                 elsif (unsigned(read_linear_addr_i(C_S_AXI_LINEAR_ADDR_LEN-1 downto 15)) = 2) then
      |                     -- 'RFC_IQ_Tx_Buffer' dout
      |                     shmem_bank_out_i <= sm_RFC_IQ_Tx_Buffer_dout_i;
      |                 elsif (unsigned(read_linear_addr_i(C_S_AXI_LINEAR_ADDR_LEN-1 downto 12)) = 65) then
      |                     -- 'RFC_RSSI_Buffer' dout
      |                     shmem_bank_out_i <= sm_RFC_RSSI_Buffer_dout_i;
      |                 elsif (unsigned(read_linear_addr_i(C_S_AXI_LINEAR_ADDR_LEN-1 downto 15)) = 3) then
      |                     -- 'RFC_IQ_Rx_Buffer' dout
      |                     shmem_bank_out_i <= sm_RFC_IQ_Rx_Buffer_dout_i;
      |                 elsif (unsigned(read_linear_addr_i(C_S_AXI_LINEAR_ADDR_LEN-1 downto 15)) = 4) then
      |                     -- 'RFB_IQ_Tx_Buffer' dout
      |                     shmem_bank_out_i <= sm_RFB_IQ_Tx_Buffer_dout_i;
      |                 elsif (unsigned(read_linear_addr_i(C_S_AXI_LINEAR_ADDR_LEN-1 downto 12)) = 66) then
      |                     -- 'RFB_RSSI_Buffer' dout
      |                     shmem_bank_out_i <= sm_RFB_RSSI_Buffer_dout_i;
      |                 elsif (unsigned(read_linear_addr_i(C_S_AXI_LINEAR_ADDR_LEN-1 downto 15)) = 5) then
      |                     -- 'RFB_IQ_Rx_Buffer' dout
      |                     shmem_bank_out_i <= sm_RFB_IQ_Rx_Buffer_dout_i;
      |                 elsif (unsigned(read_linear_addr_i(C_S_AXI_LINEAR_ADDR_LEN-1 downto 15)) = 6) then
      |                     -- 'RFA_IQ_Tx_Buffer' dout
      |                     shmem_bank_out_i <= sm_RFA_IQ_Tx_Buffer_dout_i;
      |                 elsif (unsigned(read_linear_addr_i(C_S_AXI_LINEAR_ADDR_LEN-1 downto 12)) = 67) then
      |                     -- 'RFA_RSSI_Buffer' dout
      |                     shmem_bank_out_i <= sm_RFA_RSSI_Buffer_dout_i;
      |                 elsif (unsigned(read_linear_addr_i(C_S_AXI_LINEAR_ADDR_LEN-1 downto 15)) = 7) then
      |                     -- 'RFA_IQ_Rx_Buffer' dout
      |                     shmem_bank_out_i <= sm_RFA_IQ_Rx_Buffer_dout_i;
      |                 end if;
      | 
      |                 S_AXI_RDATA_i <= shmem_bank_out_i;
      |             end if;
      |         end if;
      |     end if;
      | end process Read_Linear_Addr_Decode;
      | 
      | end architecture IMP;
      settings: infoedit=For use with EDK Processor block.
  wires:
  memmap/60 -> Shared Memory11/4, Shared Memory10/4, Shared Memory9/4, Shared Memory8/4, Shared Memory7/4, Shared Memory6/4, Shared Memory5/4, Shared Memory4/4, Shared Memory3/4, Shared Memory2/4, Shared Memory1/4, Shared Memory/4
  memmap/23 -> To Register5/2
  memmap/22 -> To Register5/1
  memmap/13 -> To Register/2
  memmap/12 -> To Register/1
  memmap/19 -> To Register3/2
  memmap/18 -> To Register3/1
  memmap/21 -> To Register4/2
  memmap/20 -> To Register4/1
  memmap/15 -> To Register1/2
  memmap/14 -> To Register1/1
  memmap/29 -> Shared Memory1/3
  memmap/28 -> Shared Memory1/2
  memmap/27 -> Shared Memory1/1
  memmap/26 -> Shared Memory/3
  memmap/25 -> Shared Memory/2
  memmap/24 -> Shared Memory/1
  memmap/32 -> Shared Memory2/3
  memmap/31 -> Shared Memory2/2
  memmap/30 -> Shared Memory2/1
  memmap/38 -> Shared Memory4/3
  memmap/37 -> Shared Memory4/2
  memmap/36 -> Shared Memory4/1
  memmap/35 -> Shared Memory3/3
  memmap/34 -> Shared Memory3/2
  memmap/33 -> Shared Memory3/1
  memmap/41 -> Shared Memory5/3
  memmap/40 -> Shared Memory5/2
  memmap/39 -> Shared Memory5/1
  memmap/47 -> Shared Memory7/3
  memmap/46 -> Shared Memory7/2
  memmap/45 -> Shared Memory7/1
  memmap/44 -> Shared Memory6/3
  memmap/43 -> Shared Memory6/2
  memmap/42 -> Shared Memory6/1
  memmap/50 -> Shared Memory8/3
  memmap/49 -> Shared Memory8/2
  memmap/48 -> Shared Memory8/1
  memmap/56 -> Shared Memory10/3
  memmap/55 -> Shared Memory10/2
  memmap/54 -> Shared Memory10/1
  memmap/53 -> Shared Memory9/3
  memmap/52 -> Shared Memory9/2
  memmap/51 -> Shared Memory9/1
  memmap/59 -> Shared Memory11/3
  memmap/58 -> Shared Memory11/2
  memmap/57 -> Shared Memory11/1
  memmap/17 -> To Register2/2
  memmap/16 -> To Register2/1
  memmap/11 -> S_AXI_WREADY/1
  memmap/10 -> S_AXI_RVALID/1
  memmap/9 -> S_AXI_RRESP/1
  memmap/8 -> S_AXI_RLAST/1
  memmap/7 -> S_AXI_RID/1
  memmap/6 -> S_AXI_RDATA/1
  memmap/5 -> S_AXI_BVALID/1
  memmap/4 -> S_AXI_BRESP/1
  memmap/3 -> S_AXI_BID/1
  memmap/2 -> S_AXI_AWREADY/1
  memmap/1 -> S_AXI_ARREADY/1
  S_AXI_WVALID/1 -> memmap/25
  S_AXI_WSTRB/1 -> memmap/24
  S_AXI_WLAST/1 -> memmap/23
  S_AXI_WDATA/1 -> memmap/22
  S_AXI_RREADY/1 -> memmap/21
  S_AXI_BREADY/1 -> memmap/20
  S_AXI_AWVALID/1 -> memmap/19
  S_AXI_AWSIZE/1 -> memmap/18
  S_AXI_AWPROT/1 -> memmap/17
  S_AXI_AWLOCK/1 -> memmap/16
  S_AXI_AWLEN/1 -> memmap/15
  S_AXI_AWID/1 -> memmap/14
  S_AXI_AWCACHE/1 -> memmap/13
  S_AXI_AWBURST/1 -> memmap/12
  S_AXI_AWADDR/1 -> memmap/11
  S_AXI_ARVALID/1 -> memmap/10
  S_AXI_ARSIZE/1 -> memmap/9
  S_AXI_ARPROT/1 -> memmap/8
  S_AXI_ARLOCK/1 -> memmap/7
  S_AXI_ARLEN/1 -> memmap/6
  S_AXI_ARID/1 -> memmap/5
  S_AXI_ARCACHE/1 -> memmap/4
  S_AXI_ARBURST/1 -> memmap/3
  S_AXI_ARADDR/1 -> memmap/2
  AXI_ARESETN/1 -> memmap/1
  To Register5/1 -> memmap/37
  To Register/1 -> memmap/32
  To Register3/1 -> memmap/35
  From Register2/1 -> memmap/28
  To Register4/1 -> memmap/36
  To Register1/1 -> memmap/33
  Shared Memory1/1 -> memmap/39
  Shared Memory/1 -> memmap/38
  Shared Memory2/1 -> memmap/40
  Shared Memory4/1 -> memmap/42
  Shared Memory3/1 -> memmap/41
  Shared Memory5/1 -> memmap/43
  From Register3/1 -> memmap/29
  Shared Memory7/1 -> memmap/45
  Shared Memory6/1 -> memmap/44
  Shared Memory8/1 -> memmap/46
  Shared Memory10/1 -> memmap/48
  Shared Memory9/1 -> memmap/47
  Shared Memory11/1 -> memmap/49
  From Register4/1 -> memmap/30
  From Register1/1 -> memmap/27
  To Register2/1 -> memmap/34
  From Register/1 -> memmap/26
  From Register5/1 -> memmap/31
  S_AXI_WREADY/1 -> Terminator10/1
  S_AXI_RVALID/1 -> Terminator9/1
  S_AXI_RRESP/1 -> Terminator8/1
  S_AXI_RLAST/1 -> Terminator7/1
  S_AXI_RID/1 -> Terminator6/1
  S_AXI_RDATA/1 -> Terminator5/1
  S_AXI_BVALID/1 -> Terminator4/1
  S_AXI_BRESP/1 -> Terminator3/1
  S_AXI_BID/1 -> Terminator2/1
  S_AXI_AWREADY/1 -> Terminator1/1
  S_AXI_ARREADY/1 -> Terminator/1
  Constant24/1 -> S_AXI_WVALID/1
  Constant23/1 -> S_AXI_WSTRB/1
  Constant22/1 -> S_AXI_WLAST/1
  Constant21/1 -> S_AXI_WDATA/1
  Constant20/1 -> S_AXI_RREADY/1
  Constant19/1 -> S_AXI_BREADY/1
  Constant18/1 -> S_AXI_AWVALID/1
  Constant17/1 -> S_AXI_AWSIZE/1
  Constant16/1 -> S_AXI_AWPROT/1
  Constant15/1 -> S_AXI_AWLOCK/1
  Constant14/1 -> S_AXI_AWLEN/1
  Constant13/1 -> S_AXI_AWID/1
  Constant12/1 -> S_AXI_AWCACHE/1
  Constant11/1 -> S_AXI_AWBURST/1
  Constant10/1 -> S_AXI_AWADDR/1
  Constant9/1 -> S_AXI_ARVALID/1
  Constant8/1 -> S_AXI_ARSIZE/1
  Constant7/1 -> S_AXI_ARPROT/1
  Constant6/1 -> S_AXI_ARLOCK/1
  Constant5/1 -> S_AXI_ARLEN/1
  Constant4/1 -> S_AXI_ARID/1
  Constant3/1 -> S_AXI_ARCACHE/1
  Constant2/1 -> S_AXI_ARBURST/1
  Constant1/1 -> S_AXI_ARADDR/1
  Constant/1 -> AXI_ARESETN/1
